simulink library "xbsIndex_r4"  (Simulink 7.1)
(part 4 of 9)

  Expression : S-Function  LoadFcn=xlBlockLoadCallback(gcbh);  FunctionName=sysgen  Parameters=ptable_  EnableBusSupport=off  mask(Xilinx Bitwise Expression Evaluator Block){expression=a & b, align_bp_sgadvanced=, align_bp=on, en_sgadvanced=, en=off, latency=0, precision_sgadvanced=, precision=Full, arith_type_sgadvanced=, arith_type=Unsigned, n_bits=16, bin_pt=0, dbl_ovrd_sgadvanced=, dbl_ovrd=off, xl_use_area_sgadvanced=, xl_use_area=off, xl_area=[0,0,0,0,0,0,0], has_advanced_control=0, sggui_pos=-1,-1,-1,-1, block_type=expr, block_version=, sg_icon_stat=65,60,2,1,white,blue,0,87655dbc,right,,[ ],[ ], sg_mask_display=|, sg_list_contents=, sg_blockgui_xml=}
      mask sg_mask_display=|
      | fprintf('','COMMENT: begin icon graphics');
      | patch([0 65 65 0 0 ],[0 0 60 60 0 ],[0.77 0.82 0.91 ]);
      | plot([0 65 65 0 0 ],[0 0 60 60 0 ]);
      | patch([14.2 25.76 33.76 41.76 49.76 33.76 22.2 14.2 ],[38.88 38.88 46.88 38.88 46.88 46.88 46.88 38.88 ],[1 1 1 ]);
      | patch([22.2 33.76 25.76 14.2 22.2 ],[30.88 30.88 38.88 38.88 30.88 ],[0.931 0.946 0.973 ]);
      | patch([14.2 25.76 33.76 22.2 14.2 ],[22.88 22.88 30.88 30.88 22.88 ],[1 1 1 ]);
      | patch([22.2 49.76 41.76 33.76 25.76 14.2 22.2 ],[14.88 14.88 22.88 14.88 22.88 22.88 14.88 ],[0.931 0.946 0.973 ]);
      | fprintf('','COMMENT: end icon graphics');
      | fprintf('','COMMENT: begin icon text');
      | color('black');port_label('input',1,'a');
      | color('black');port_label('input',2,'b');
      | color('black');port_label('output',1,'\bfa & b','texmode','on');
      | fprintf('','COMMENT: end icon text');
      mask prompts: align_bp_sgadvanced ""; align_bp "Align binary point"; en_sgadvanced ""; en "Provide enable port"; precision_sgadvanced ""; arith_type_sgadvanced ""; arith_type "Arithmetic type"; n_bits "Number of bits"; bin_pt "Binary point"; dbl_ovrd_sgadvanced ""; dbl_ovrd "Override with doubles"; xl_use_area_sgadvanced ""; xl_use_area "Define FPGA area for resource estimation"; xl_area "FPGA area [slices, FFs, BRAMs, LUTs, IOBs, emb. mults, TBUFs]"; has_advanced_control ""; sggui_pos ""; block_type ""; block_version ""; sg_icon_stat ""; sg_mask_display ""; sg_list_contents ""; sg_blockgui_xml ""
      mask help: Xilinx Bitwise Expression Evaluator
      mask init:
      | try
      |   tmp_gcb = gcb;
      |   tmp_gcbh = gcbh;
      |   if (strcmp('SysGenIndex',get_param(bdroot(tmp_gcbh),'tag')) && ~isempty(regexp(bdroot(tmp_gcb), '^xbs', 'once')))
      |     return;
      |   end;
      |   xlMungeMaskParams;
      |   block_config = 'sysgen_blockset:Expr_config';
      | 
      |   block_type='expr';
      | 
      |   serialized_declarations = '{''align_bp''=>''Int'',''arith_type''=>''Int'',''bin_pt''=>''Int'',''dbl_ovrd''=>''Int'',''en''=>''Int'',''expression''=>''String'',''inports''=>''String'',''latency''=>''Int'',''n_bits''=>''Int'',''period''=>''Double'',''precision''=>''Int'',''sim_engine''=>''Int'',''sysgen_root''=>''String'',''block_type''=>''String''}';
      |   xlexpr_init();
      |   ptable_ = xlblockprep(get_param(tmp_gcb, 'MaskWSVariables'));
      |   try
      |     xlBlockMoveCallback(tmp_gcbh);
      |   catch 
      |      clear global xl_updateicon_recursion_guard;
      |   end;
      | catch
      |   global dbgsysgen;
      |   if(~isempty(dbgsysgen) && dbgsysgen)
      |     e = regexprep(lasterr, '\n', '\nError: ');
      |     disp(['Error: While running MaskInit code on block ' tmp_gcb ': ' e]);
      |     error(e);
      |   end
      | end
      settings: CopyFcn=xlBlockMoveCallback(gcbh);  DeleteFcn=xlDestroyGui(gcbh);  ModelCloseFcn=xlDestroyGui(gcbh);  PreSaveFcn=xlBlockPreSaveCallback(gcbh);  PostSaveFcn=xlBlockPostSaveCallback(gcbh);  DestroyFcn=xlDestroyGui(gcbh);  OpenFcn=xlOpenGui(gcbh, 'expr_gui.xml', @xlmagicenablement, -1)  CloseFcn=xlDestroyGui(gcbh);  MoveFcn=xlBlockMoveCallback(gcbh);
      mask Help: eval('');xlDoc('-book','sysgen','-topic','Expression');
      mask StyleString: edit,edit,checkbox,edit,checkbox,edit,edit,popup(Full|User Defined),edit,popup(Signed  (2's comp)|Unsigned),edit,edit,edit,checkbox,edit,checkbox,edit,edit,edit,edit,edit,edit,edit,edit,edit
      mask Display:
      | fprintf('','COMMENT: begin icon graphics');
      | patch([0 65 65 0 0 ],[0 0 60 60 0 ],[0.77 0.82 0.91 ]);
      | plot([0 65 65 0 0 ],[0 0 60 60 0 ]);
      | patch([14.2 25.76 33.76 41.76 49.76 33.76 22.2 14.2 ],[38.88 38.88 46.88 38.88 46.88 46.88 46.88 38.88 ],[1 1 1 ]);
      | patch([22.2 33.76 25.76 14.2 22.2 ],[30.88 30.88 38.88 38.88 30.88 ],[0.931 0.946 0.973 ]);
      | patch([14.2 25.76 33.76 22.2 14.2 ],[22.88 22.88 30.88 30.88 22.88 ],[1 1 1 ]);
      | patch([22.2 49.76 41.76 33.76 25.76 14.2 22.2 ],[14.88 14.88 22.88 14.88 22.88 22.88 14.88 ],[0.931 0.946 0.973 ]);
      | fprintf('','COMMENT: end icon graphics');
      | fprintf('','COMMENT: begin icon text');
      | color('black');port_label('input',1,'a');
      | color('black');port_label('input',2,'b');
      | color('black');port_label('output',1,'\bfa & b','texmode','on');
      | fprintf('','COMMENT: end icon text');
  FDATool : S-Function  FunctionName=xlpermissive  Parameters=''  EnableBusSupport=off  mask(Xilinx FDATool Interface Block){infoedit=FDATool, ShowPortLabels=, has_advanced_control=0, sggui_pos=-1,-1,-1,-1, block_type=fdatool, block_version=, sg_icon_stat=54,56,-1,-1,blue,white,0,07734,right,,[ ],[ ], sg_mask_display=|, sg_list_contents=, sg_blockgui_xml=}
      mask sg_mask_display=|
      | fprintf('','COMMENT: begin icon graphics');
      | patch([0 54 54 0 0 ],[0 0 56 56 0 ],[1 1 1 ]);
      | plot([0 54 54 0 0 ],[0 0 56 56 0 ]);
      | patch([11.425 21.54 28.54 35.54 42.54 28.54 18.425 11.425 ],[35.77 35.77 42.77 35.77 42.77 42.77 42.77 35.77 ],[0.839 0.874 0.937 ]);
      | patch([18.425 28.54 21.54 11.425 18.425 ],[28.77 28.77 35.77 35.77 28.77 ],[0.77 0.82 0.91 ]);
      | patch([11.425 21.54 28.54 18.425 11.425 ],[21.77 21.77 28.77 28.77 21.77 ],[0.839 0.874 0.937 ]);
      | patch([18.425 42.54 35.54 28.54 21.54 11.425 18.425 ],[14.77 14.77 21.77 14.77 21.77 21.77 14.77 ],[0.77 0.82 0.91 ]);
      | fprintf('','COMMENT: end icon graphics');
      | fprintf('','COMMENT: begin icon text');
      | fprintf('','COMMENT: end icon text');plot(foox,foo);
      mask prompts: infoedit ""; ShowPortLabels ""; has_advanced_control ""; sggui_pos ""; block_type ""; block_version ""; sg_icon_stat ""; sg_mask_display ""; sg_list_contents ""; sg_blockgui_xml ""
      mask help: FDATool
      mask init:
      | try
      |   tmp_gcb = gcb;
      |   tmp_gcbh = gcbh;
      |   xlMungeMaskParams;
      | 
      |   block_type='fdatool';
      | 
      |   serialized_declarations = '{''block_type''=>''String''}';
      |   xlfdatool_init();
      |   ptable_ = xlblockprep(get_param(tmp_gcb, 'MaskWSVariables'));
      |   try
      |     xlBlockMoveCallback(tmp_gcbh);
      |   catch 
      |      clear global xl_updateicon_recursion_guard;
      |   end;
      | catch
      |   global dbgsysgen;
      |   if(~isempty(dbgsysgen) && dbgsysgen)
      |     e = regexprep(lasterr, '\n', '\nError: ');
      |     disp(['Error: While running MaskInit code on block ' tmp_gcb ': ' e]);
      |     error(e);
      |   end
      | end
      settings: CopyFcn=xlfdatool_utils('BlockCopy');  DeleteFcn=xlfdatool_utils('CloseFcn');  ModelCloseFcn=xlfdatool_utils('ModelCloseFcn');  NameChangeFcn=xlfdatool_utils('NameChange');  OpenFcn=xlfdatool_utils('OpenFcn');  CloseFcn=xlfdatool_utils('CloseFcn');  MoveFcn=xlBlockMoveCallback(gcbh);
      mask Help: eval('');xlDoc('-book','sysgen','-topic','FDATool');
      mask Display:
      | fprintf('','COMMENT: begin icon graphics');
      | patch([0 54 54 0 0 ],[0 0 56 56 0 ],[1 1 1 ]);
      | plot([0 54 54 0 0 ],[0 0 56 56 0 ]);
      | patch([11.425 21.54 28.54 35.54 42.54 28.54 18.425 11.425 ],[35.77 35.77 42.77 35.77 42.77 42.77 42.77 35.77 ],[0.839 0.874 0.937 ]);
      | patch([18.425 28.54 21.54 11.425 18.425 ],[28.77 28.77 35.77 35.77 28.77 ],[0.77 0.82 0.91 ]);
      | patch([11.425 21.54 28.54 18.425 11.425 ],[21.77 21.77 28.77 28.77 21.77 ],[0.839 0.874 0.937 ]);
      | patch([18.425 42.54 35.54 28.54 21.54 11.425 18.425 ],[14.77 14.77 21.77 14.77 21.77 21.77 14.77 ],[0.77 0.82 0.91 ]);
      | fprintf('','COMMENT: end icon graphics');
      | fprintf('','COMMENT: begin icon text');
      | fprintf('','COMMENT: end icon text');plot(foox,foo);
  "FFT v1_0 " : S-Function  LoadFcn=xlBlockLoadCallback(gcbh);  FunctionName=sysgen  Parameters=ptable_  EnableBusSupport=off  mask(Xilinx Fast Fourier Transform v1_0 Block){infoedit=Radix-4 Cooley-Tukey fast Fourier transform (FFT).  Supports 16, 64, 256, and 1024 point transforms on 16-bit data.<br><br>Devices Supported: Virtex, n_sgadvanced=, n=64, mem_sgadvanced=, mem=Triple, scale_mode_sgadvanced=, scale_mode=1/N, oflw_inv_sgadvanced=, oflw_inv=on, rst_sgadvanced=, rst=off, dbl_ovrd_sgadvanced=, dbl_ovrd=off, explicit_period_sgadvanced=, explicit_period=off, period=1, xl_use_area_sgadvanced=, xl_use_area=off, xl_area=[0,0,0,0,0,0,0], has_advanced_control=0, sggui_pos=-1,-1,-1,-1, block_type=fft, block_version=, sg_icon_stat=60,88,-1,-1,white,blue,0,07734,right,,[ ],[ ], sg_mask_display=|, sg_list_contents=, sg_blockgui_xml=}
      mask sg_mask_display=|
      | fprintf('','COMMENT: begin icon graphics');
      | patch([0 60 60 0 0 ],[0 0 88 88 0 ],[0.77 0.82 0.91 ]);
      | plot([0 60 60 0 0 ],[0 0 88 88 0 ]);
      | patch([12.2 23.76 31.76 39.76 47.76 31.76 20.2 12.2 ],[52.88 52.88 60.88 52.88 60.88 60.88 60.88 52.88 ],[1 1 1 ]);
      | patch([20.2 31.76 23.76 12.2 20.2 ],[44.88 44.88 52.88 52.88 44.88 ],[0.931 0.946 0.973 ]);
      | patch([12.2 23.76 31.76 20.2 12.2 ],[36.88 36.88 44.88 44.88 36.88 ],[1 1 1 ]);
      | patch([20.2 47.76 39.76 31.76 23.76 12.2 20.2 ],[28.88 28.88 36.88 28.88 36.88 36.88 28.88 ],[0.931 0.946 0.973 ]);
      | fprintf('','COMMENT: end icon graphics');
      | fprintf('','COMMENT: begin icon text');
      | fprintf('','COMMENT: end icon text');
      mask prompts: infoedit ""; n_sgadvanced ""; n "Number of sample points (N)"; mem_sgadvanced ""; mem "Memory usage"; scale_mode_sgadvanced ""; scale_mode "Scale output by"; oflw_inv_sgadvanced ""; oflw_inv "Invalidate transform on overflow"; rst_sgadvanced ""; rst "Provide synchronous reset port"; dbl_ovrd_sgadvanced ""; dbl_ovrd "Override with doubles"; explicit_period_sgadvanced ""; explicit_period "Specify explicit sample period"; period ""; xl_use_area_sgadvanced ""; xl_use_area "Define FPGA area for resource estimation"; xl_area "FPGA area [slices, FFs, BRAMs, LUTs, IOBs, emb. mults, TBUFs]"; has_advanced_control ""; sggui_pos ""; block_type ""; block_version ""; sg_icon_stat ""; sg_mask_display ""; sg_list_contents ""; sg_blockgui_xml ""
      mask help:
      | Radix-4 Cooley-Tukey fast Fourier transform (FFT).  Supports 16, 64, 256, and 1024 point transforms on 16-bit data.
      |
      | Devices Supported: Virtex
      mask init:
      | try
      |   tmp_gcb = gcb;
      |   tmp_gcbh = gcbh;
      |   if (strcmp('SysGenIndex',get_param(bdroot(tmp_gcbh),'tag')) && ~isempty(regexp(bdroot(tmp_gcb), '^xbs', 'once')))
      |     return;
      |   end;
      |   xlMungeMaskParams;
      |   block_config = 'sysgen_blockset:Removed_config';
      | 
      |   block_type='fft';
      | nport = get_param(gcbh, 'ports');
      | nin = nport(1);
      | nout = nport(2);
      | 
      |   serialized_declarations = '{''memory_usage''=>''Int'',''npts''=>''Int'',''oflw_inv''=>''Int'',''period''=>''Double'',''scale_mode''=>''Int'',''block_type''=>''String'',''nin''=>''Double'',''nout''=>''Double''}';
      |   xlfft_init();
      |   ptable_ = xlblockprep(get_param(tmp_gcb, 'MaskWSVariables'));
      |   try
      |     xlBlockMoveCallback(tmp_gcbh);
      |   catch 
      |      clear global xl_updateicon_recursion_guard;
      |   end;
      | catch
      |   global dbgsysgen;
      |   if(~isempty(dbgsysgen) && dbgsysgen)
      |     e = regexprep(lasterr, '\n', '\nError: ');
      |     disp(['Error: While running MaskInit code on block ' tmp_gcb ': ' e]);
      |     error(e);
      |   end
      | end
      settings: CopyFcn=xlBlockMoveCallback(gcbh);  DeleteFcn=xlDestroyGui(gcbh);  ModelCloseFcn=xlDestroyGui(gcbh);  PreSaveFcn=xlBlockPreSaveCallback(gcbh);  PostSaveFcn=xlBlockPostSaveCallback(gcbh);  DestroyFcn=xlDestroyGui(gcbh);  OpenFcn=xlOpenGui(gcbh, 'fft_gui.xml', @xlremovedenablement, -1)  CloseFcn=xlDestroyGui(gcbh);  MoveFcn=xlBlockMoveCallback(gcbh);
      mask Help: eval('');xlDoc('-book','sysgen','-topic','FFT_v1_0');
      mask StyleString: edit,edit,popup(16|64|256|1024),edit,popup(Single|Double|Triple),edit,popup(1/N|1/(2N)),edit,checkbox,edit,checkbox,edit,checkbox,edit,checkbox,edit,edit,checkbox,edit,edit,edit,edit,edit,edit,edit,edit,edit
      mask Display:
      | fprintf('','COMMENT: begin icon graphics');
      | patch([0 60 60 0 0 ],[0 0 88 88 0 ],[0.77 0.82 0.91 ]);
      | plot([0 60 60 0 0 ],[0 0 88 88 0 ]);
      | patch([12.2 23.76 31.76 39.76 47.76 31.76 20.2 12.2 ],[52.88 52.88 60.88 52.88 60.88 60.88 60.88 52.88 ],[1 1 1 ]);
      | patch([20.2 31.76 23.76 12.2 20.2 ],[44.88 44.88 52.88 52.88 44.88 ],[0.931 0.946 0.973 ]);
      | patch([12.2 23.76 31.76 20.2 12.2 ],[36.88 36.88 44.88 44.88 36.88 ],[1 1 1 ]);
      | patch([20.2 47.76 39.76 31.76 23.76 12.2 20.2 ],[28.88 28.88 36.88 28.88 36.88 36.88 28.88 ],[0.931 0.946 0.973 ]);
      | fprintf('','COMMENT: end icon graphics');
      | fprintf('','COMMENT: begin icon text');
      | fprintf('','COMMENT: end icon text');
  "FFT v3_1 " : S-Function  LoadFcn=xlBlockLoadCallback(gcbh);  FunctionName=sysgen  Parameters=ptable_  EnableBusSupport=off  mask(Xilinx Fast Fourier Transform v3_1 Block){infoedit=Devices Supported: Virtex-4, Virtex-II, Virtex-IIPro, Spartan-3 and Spartan-3E, arch_sgadvanced=, arch=Pipelined Streaming I/O, npts_sgadvanced=, npts=64, scaling_sgadvanced=, scaling=Unscaled, rounding_sgadvanced=, rounding=Truncation, tf_width_sgadvanced=, tf_width=8, en_n_sgadvanced=, en_n=off, has_ovflo_sgadvanced=, has_ovflo=off, rst_sgadvanced=, rst=off, en_sgadvanced=, en=off, op_order_sgadvanced=, op_order=Bit Reversed Order, dbl_ovrd_sgadvanced=, dbl_ovrd=off, explicit_period_sgadvanced=, explicit_period=off, period=1, use_dsp48_sgadvanced=, use_dsp48=off, twiddle_mem_type_sgadvanced=, twiddle_mem_type=Block RAM, data_mem_type_sgadvanced=, data_mem_type=Block RAM, num_bram_stages_sgadvanced=, num_bram_stages=3, xl_use_area_sgadvanced=, xl_use_area=off, xl_area=[0,0,0,0,0,0,0], has_advanced_control=0, sggui_pos=-1,-1,-1,-1, block_type=fftx, block_version=, sg_icon_stat=100,146,-1,-1,white,blue,0,07734,right,,[ ],[ ], sg_mask_display=|, sg_list_contents=, sg_blockgui_xml=}
      mask sg_mask_display=|
      | fprintf('','COMMENT: begin icon graphics');
      | patch([0 100 100 0 0 ],[0 0 146 146 0 ],[0.77 0.82 0.91 ]);
      | plot([0 100 100 0 0 ],[0 0 146 146 0 ]);
      | patch([18.85 39.08 53.08 67.08 81.08 53.08 32.85 18.85 ],[88.54 88.54 102.54 88.54 102.54 102.54 102.54 88.54 ],[1 1 1 ]);
      | patch([32.85 53.08 39.08 18.85 32.85 ],[74.54 74.54 88.54 88.54 74.54 ],[0.931 0.946 0.973 ]);
      | patch([18.85 39.08 53.08 32.85 18.85 ],[60.54 60.54 74.54 74.54 60.54 ],[1 1 1 ]);
      | patch([32.85 81.08 67.08 53.08 39.08 18.85 32.85 ],[46.54 46.54 60.54 46.54 60.54 60.54 46.54 ],[0.931 0.946 0.973 ]);
      | fprintf('','COMMENT: end icon graphics');
      | fprintf('','COMMENT: begin icon text');
      | fprintf('','COMMENT: end icon text');
      mask prompts: infoedit ""; arch_sgadvanced ""; arch "Implementation"; npts_sgadvanced ""; npts "Number of sample points"; scaling_sgadvanced ""; rounding_sgadvanced ""; rounding "Rounding mode"; tf_width_sgadvanced ""; tf_width "Phase factor bit width"; en_n_sgadvanced ""; en_n "Enable dynamic transform size"; has_ovflo_sgadvanced ""; has_ovflo "Provide overflow port"; rst_sgadvanced ""; rst "Provide synchronous reset port"; en_sgadvanced ""; en "Provide enable port"; op_order_sgadvanced ""; op_order "Output ordering"; dbl_ovrd_sgadvanced ""; dbl_ovrd "Override with doubles"; explicit_period_sgadvanced ""; explicit_period "Specify explicit sample period"; period ""; use_dsp48_sgadvanced ""; use_dsp48 "Optimize for speed using DSP48"; twiddle_mem_type_sgadvanced ""; twiddle_mem_type "Phase factor memory type"; data_mem_type_sgadvanced ""; data_mem_type "Data memory type"; num_bram_stages_sgadvanced ""; num_bram_stages "Number of stages using block RAM"; xl_use_area_sgadvanced ""; xl_use_area "Define FPGA area for resource estimation"; xl_area "FPGA area [slices, FFs, BRAMs, LUTs, IOBs, emb. mults, TBUFs]"; has_advanced_control ""; sggui_pos ""; block_type ""; block_version ""; sg_icon_stat ""; sg_mask_display ""; sg_list_contents ""; sg_blockgui_xml ""
      mask help: Devices Supported: Virtex-4, Virtex-II, Virtex-IIPro, Spartan-3 and Spartan-3E
      mask init:
      | try
      |   tmp_gcb = gcb;
      |   tmp_gcbh = gcbh;
      |   if (strcmp('SysGenIndex',get_param(bdroot(tmp_gcbh),'tag')) && ~isempty(regexp(bdroot(tmp_gcb), '^xbs', 'once')))
      |     return;
      |   end;
      |   xlMungeMaskParams;
      |   block_config = 'sysgen_blockset:Removed_config';
      | 
      |   block_type='fftx';
      | nport = get_param(gcbh, 'ports');
      | nin = nport(1);
      | nout = nport(2);
      | 
      |   serialized_declarations = '{''arch''=>''Int'',''c_family''=>''Int'',''data_mem_type''=>''Int'',''en''=>''Int'',''en_n''=>''Int'',''has_ovflo''=>''Int'',''npts''=>''Int'',''num_bram_stages''=>''Int'',''op_order''=>''Int'',''period''=>''Double'',''rounding''=>''Int'',''rst''=>''Int'',''scaling''=>''Int'',''tf_width''=>''Int'',''twiddle_mem_type''=>''Int'',''use_dsp48''=>''Int'',''xlISEVer''=>''String'',''xlv2fft_dll''=>''String'',''block_type''=>''String'',''nin''=>''Double'',''nout''=>''Double''}';
      |   xlfftx_init();
      |   ptable_ = xlblockprep(get_param(tmp_gcb, 'MaskWSVariables'));
      |   try
      |     xlBlockMoveCallback(tmp_gcbh);
      |   catch 
      |      clear global xl_updateicon_recursion_guard;
      |   end;
      | catch
      |   global dbgsysgen;
      |   if(~isempty(dbgsysgen) && dbgsysgen)
      |     e = regexprep(lasterr, '\n', '\nError: ');
      |     disp(['Error: While running MaskInit code on block ' tmp_gcb ': ' e]);
      |     error(e);
      |   end
      | end
      settings: CopyFcn=xlBlockMoveCallback(gcbh);  DeleteFcn=xlDestroyGui(gcbh);  ModelCloseFcn=xlDestroyGui(gcbh);  PreSaveFcn=xlBlockPreSaveCallback(gcbh);  PostSaveFcn=xlBlockPostSaveCallback(gcbh);  DestroyFcn=xlDestroyGui(gcbh);  OpenFcn=xlOpenGui(gcbh, 'fftx_gui.xml', @xlremovedenablement, -1)  CloseFcn=xlDestroyGui(gcbh);  MoveFcn=xlBlockMoveCallback(gcbh);
      mask Help: eval('');xlDoc('-book','sysgen','-topic','FFT_v3_1');
      mask StyleString: edit,edit,popup(Radix-4 Streaming I/O|Radix-4 Burst I/O|Radix-2 Minimum Resources|Pipelined Streaming I/O),edit,popup(8|16|32|64|128|256|512|1024|2048|4096|8192|16384|32768|65536),edit,popup(Unscaled|Scaled|Block Floating Point),edit,popup(Truncation|Convergent Rounding),edit,popup(8|12|16|20|24),edit,checkbox,edit,checkbox,edit,checkbox,edit,checkbox,edit,popup(Bit Reversed Order|Natural Order),edit,checkbox,edit,checkbox,edit,edit,checkbox,edit,popup(Block RAM|Distributed RAM),edit,popup(Block RAM|Distributed RAM),edit,popup(0|1|2|3|4|5|6|7|8|9|10|11|12|13),edit,checkbox,edit,edit,edit,edit,edit,edit,edit,edit,edit
      mask Display:
      | fprintf('','COMMENT: begin icon graphics');
      | patch([0 100 100 0 0 ],[0 0 146 146 0 ],[0.77 0.82 0.91 ]);
      | plot([0 100 100 0 0 ],[0 0 146 146 0 ]);
      | patch([18.85 39.08 53.08 67.08 81.08 53.08 32.85 18.85 ],[88.54 88.54 102.54 88.54 102.54 102.54 102.54 88.54 ],[1 1 1 ]);
      | patch([32.85 53.08 39.08 18.85 32.85 ],[74.54 74.54 88.54 88.54 74.54 ],[0.931 0.946 0.973 ]);
      | patch([18.85 39.08 53.08 32.85 18.85 ],[60.54 60.54 74.54 74.54 60.54 ],[1 1 1 ]);
      | patch([32.85 81.08 67.08 53.08 39.08 18.85 32.85 ],[46.54 46.54 60.54 46.54 60.54 60.54 46.54 ],[0.931 0.946 0.973 ]);
      | fprintf('','COMMENT: end icon graphics');
      | fprintf('','COMMENT: begin icon text');
      | fprintf('','COMMENT: end icon text');
  "FFT v3_2 " : S-Function  LoadFcn=xlBlockLoadCallback(gcbh);  FunctionName=sysgen  Parameters=ptable_  EnableBusSupport=off  mask(Xilinx Fast Fourier Transform v3_2 Block){infoedit=Devices Supported: Virtex-4, Virtex-II, Virtex-IIPro, Spartan-3 and Spartan-3E, arch_sgadvanced=, arch=Pipelined Streaming I/O, npts_sgadvanced=, npts=1024, op_order_sgadvanced=, op_order=Natural Order, scaling_sgadvanced=, scaling=Unscaled, rounding_sgadvanced=, rounding=Truncation, tf_width_sgadvanced=, tf_width=8, en_n_sgadvanced=, en_n=off, has_ovflo_sgadvanced=, has_ovflo=off, rst_sgadvanced=, rst=off, en_sgadvanced=, en=off, dbl_ovrd_sgadvanced=, dbl_ovrd=off, use_dsp48_bfly_sgadvanced=, use_dsp48_bfly=off, use_dsp48_cmpy_sgadvanced=, use_dsp48_cmpy=off, use_dsp48_sincos_sgadvanced=, use_dsp48_sincos=off, twiddle_mem_type_sgadvanced=, twiddle_mem_type=Block RAM, data_mem_type_sgadvanced=, data_mem_type=Block RAM, num_bram_stages_sgadvanced=, num_bram_stages=3, xl_use_area_sgadvanced=, xl_use_area=off, xl_area=[0,0,0,0,0,0,0], explicit_period=, period=1, has_advanced_control=0, sggui_pos=-1,-1,-1,-1, block_type=fftv32, block_version=, sg_icon_stat=100,146,-1,-1,white,blue,0,07734,right,,[ ],[ ], sg_mask_display=|, sg_list_contents=, sg_blockgui_xml=}
      mask sg_mask_display=|
      | fprintf('','COMMENT: begin icon graphics');
      | patch([0 100 100 0 0 ],[0 0 146 146 0 ],[0.77 0.82 0.91 ]);
      | plot([0 100 100 0 0 ],[0 0 146 146 0 ]);
      | patch([18.85 39.08 53.08 67.08 81.08 53.08 32.85 18.85 ],[88.54 88.54 102.54 88.54 102.54 102.54 102.54 88.54 ],[1 1 1 ]);
      | patch([32.85 53.08 39.08 18.85 32.85 ],[74.54 74.54 88.54 88.54 74.54 ],[0.931 0.946 0.973 ]);
      | patch([18.85 39.08 53.08 32.85 18.85 ],[60.54 60.54 74.54 74.54 60.54 ],[1 1 1 ]);
      | patch([32.85 81.08 67.08 53.08 39.08 18.85 32.85 ],[46.54 46.54 60.54 46.54 60.54 60.54 46.54 ],[0.931 0.946 0.973 ]);
      | fprintf('','COMMENT: end icon graphics');
      | fprintf('','COMMENT: begin icon text');
      | fprintf('','COMMENT: end icon text');
      mask prompts: infoedit ""; arch_sgadvanced ""; arch "Implementation"; npts_sgadvanced ""; npts "Number of sample points"; op_order_sgadvanced ""; op_order "Output ordering"; scaling_sgadvanced ""; rounding_sgadvanced ""; rounding "Rounding mode"; tf_width_sgadvanced ""; tf_width "Phase factor bit width"; en_n_sgadvanced ""; en_n "Enable dynamic transform size"; has_ovflo_sgadvanced ""; has_ovflo "Provide overflow port"; rst_sgadvanced ""; rst "Provide synchronous reset port"; en_sgadvanced ""; en "Provide enable port"; dbl_ovrd_sgadvanced ""; dbl_ovrd "Override with doubles"; use_dsp48_bfly_sgadvanced ""; use_dsp48_bfly "Butterfly arithmetic"; use_dsp48_cmpy_sgadvanced ""; use_dsp48_cmpy "Complex multiplication"; use_dsp48_sincos_sgadvanced ""; use_dsp48_sincos "Phase factor generation"; twiddle_mem_type_sgadvanced ""; twiddle_mem_type "Phase factor memory type"; data_mem_type_sgadvanced ""; data_mem_type "Data memory type"; num_bram_stages_sgadvanced ""; num_bram_stages "Number of stages using block RAM"; xl_use_area_sgadvanced ""; xl_use_area "Define FPGA area for resource estimation"; xl_area "FPGA area [slices, FFs, BRAMs, LUTs, IOBs, emb. mults, TBUFs]"; explicit_period ""; period ""; has_advanced_control ""; sggui_pos ""; block_type ""; block_version ""; sg_icon_stat ""; sg_mask_display ""; sg_list_contents ""; sg_blockgui_xml ""
      mask help: Devices Supported: Virtex-4, Virtex-II, Virtex-IIPro, Spartan-3 and Spartan-3E
      mask init:
      | try
      |   tmp_gcb = gcb;
      |   tmp_gcbh = gcbh;
      |   if (strcmp('SysGenIndex',get_param(bdroot(tmp_gcbh),'tag')) && ~isempty(regexp(bdroot(tmp_gcb), '^xbs', 'once')))
      |     return;
      |   end;
      |   xlMungeMaskParams;
      |   block_config = 'sysgen_blockset:Removed_config';
      | 
      |   block_type='fftv32';
      | nport = get_param(gcbh, 'ports');
      | nin = nport(1);
      | nout = nport(2);
      | 
      |   serialized_declarations = '{''arch''=>''Int'',''c_family''=>''Int'',''data_mem_type''=>''Int'',''en''=>''Int'',''en_n''=>''Int'',''has_ovflo''=>''Int'',''npts''=>''Int'',''num_bram_stages''=>''Int'',''op_order''=>''Int'',''rounding''=>''Int'',''rst''=>''Int'',''scaling''=>''Int'',''tf_width''=>''Int'',''twiddle_mem_type''=>''Int'',''use_dsp48_bfly''=>''Int'',''use_dsp48_cmpy''=>''Int'',''use_dsp48_sincos''=>''Int'',''xlISEVer''=>''String'',''xlv3fft_dll''=>''String'',''block_type''=>''String'',''nin''=>''Double'',''nout''=>''Double''}';
      |   xlfftv32_init();
      |   ptable_ = xlblockprep(get_param(tmp_gcb, 'MaskWSVariables'));
      |   try
      |     xlBlockMoveCallback(tmp_gcbh);
      |   catch 
      |      clear global xl_updateicon_recursion_guard;
      |   end;
      | catch
      |   global dbgsysgen;
      |   if(~isempty(dbgsysgen) && dbgsysgen)
      |     e = regexprep(lasterr, '\n', '\nError: ');
      |     disp(['Error: While running MaskInit code on block ' tmp_gcb ': ' e]);
      |     error(e);
      |   end
      | end
      settings: CopyFcn=xlBlockMoveCallback(gcbh);  DeleteFcn=xlDestroyGui(gcbh);  ModelCloseFcn=xlDestroyGui(gcbh);  PreSaveFcn=xlBlockPreSaveCallback(gcbh);  PostSaveFcn=xlBlockPostSaveCallback(gcbh);  DestroyFcn=xlDestroyGui(gcbh);  OpenFcn=xlOpenGui(gcbh, 'fftv32_gui.xml', @xlremovedenablement, -1)  CloseFcn=xlDestroyGui(gcbh);  MoveFcn=xlBlockMoveCallback(gcbh);
      mask Help: eval('');xlDoc('-book','sysgen','-topic','FFT_v3_2');
      mask StyleString: edit,edit,popup(Radix-4 Burst I/O|Radix-2 Minimum Resources|Pipelined Streaming I/O),edit,popup(8|16|32|64|128|256|512|1024|2048|4096|8192|16384|32768|65536),edit,popup(Bit Reversed Order|Natural Order),edit,popup(Unscaled|Scaled|Block Floating Point),edit,popup(Truncation|Convergent Rounding),edit,popup(8|9|10|11|12|13|14|15|16|17|18|19|20|21|22|23|24),edit,checkbox,edit,checkbox,edit,checkbox,edit,checkbox,edit,checkbox,edit,checkbox,edit,checkbox,edit,checkbox,edit,popup(Block RAM|Distributed RAM),edit,popup(Block RAM|Distributed RAM),edit,popup(0|1|2|3|4|5|6|7|8|9|10|11|12|13),edit,checkbox,edit,edit,edit,edit,edit,edit,edit,edit,edit,edit,edit
      mask Display:
      | fprintf('','COMMENT: begin icon graphics');
      | patch([0 100 100 0 0 ],[0 0 146 146 0 ],[0.77 0.82 0.91 ]);
      | plot([0 100 100 0 0 ],[0 0 146 146 0 ]);
      | patch([18.85 39.08 53.08 67.08 81.08 53.08 32.85 18.85 ],[88.54 88.54 102.54 88.54 102.54 102.54 102.54 88.54 ],[1 1 1 ]);
      | patch([32.85 53.08 39.08 18.85 32.85 ],[74.54 74.54 88.54 88.54 74.54 ],[0.931 0.946 0.973 ]);
      | patch([18.85 39.08 53.08 32.85 18.85 ],[60.54 60.54 74.54 74.54 60.54 ],[1 1 1 ]);
      | patch([32.85 81.08 67.08 53.08 39.08 18.85 32.85 ],[46.54 46.54 60.54 46.54 60.54 60.54 46.54 ],[0.931 0.946 0.973 ]);
      | fprintf('','COMMENT: end icon graphics');
      | fprintf('','COMMENT: begin icon text');
      | fprintf('','COMMENT: end icon text');
  "FFT v4_1 " : S-Function  LoadFcn=xlBlockLoadCallback(gcbh);  FunctionName=sysgen  Parameters=ptable_  EnableBusSupport=off  mask(Xilinx Fast Fourier Transform v4_1 Block){infoedit=Devices Supported: Virtex-5, Virtex-4, Virtex-IIPro, Spartan-3, Spartan-3A and Spartan-3E, arch_sgadvanced=, arch=Pipelined Streaming I/O, npts_sgadvanced=, npts=1024, op_order_sgadvanced=, op_order=Natural Order, scaling_sgadvanced=, scaling=Unscaled, rounding_sgadvanced=, rounding=Truncation, tf_width_sgadvanced=, tf_width=8, en_n_sgadvanced=, en_n=off, has_ovflo_sgadvanced=, has_ovflo=off, rst_sgadvanced=, rst=off, en_sgadvanced=, en=off, dbl_ovrd_sgadvanced=, dbl_ovrd=off, use_dsp48_bfly_sgadvanced=, use_dsp48_bfly=off, use_dsp48_cmpy_sgadvanced=, use_dsp48_cmpy=off, twiddle_mem_type_sgadvanced=, twiddle_mem_type=Block RAM, data_mem_type_sgadvanced=, data_mem_type=Block RAM, num_bram_stages_sgadvanced=, num_bram_stages=3, xl_use_area_sgadvanced=, xl_use_area=off, xl_area=[0,0,0,0,0,0,0], explicit_period=, period=1, has_advanced_control=0, sggui_pos=-1,-1,-1,-1, block_type=fftv41, block_version=, sg_icon_stat=100,146,-1,-1,white,blue,0,07734,right,,[ ],[ ], sg_mask_display=|, sg_list_contents=, sg_blockgui_xml=}
      mask sg_mask_display=|
      | fprintf('','COMMENT: begin icon graphics');
      | patch([0 100 100 0 0 ],[0 0 146 146 0 ],[0.77 0.82 0.91 ]);
      | plot([0 100 100 0 0 ],[0 0 146 146 0 ]);
      | patch([18.85 39.08 53.08 67.08 81.08 53.08 32.85 18.85 ],[88.54 88.54 102.54 88.54 102.54 102.54 102.54 88.54 ],[1 1 1 ]);
      | patch([32.85 53.08 39.08 18.85 32.85 ],[74.54 74.54 88.54 88.54 74.54 ],[0.931 0.946 0.973 ]);
      | patch([18.85 39.08 53.08 32.85 18.85 ],[60.54 60.54 74.54 74.54 60.54 ],[1 1 1 ]);
      | patch([32.85 81.08 67.08 53.08 39.08 18.85 32.85 ],[46.54 46.54 60.54 46.54 60.54 60.54 46.54 ],[0.931 0.946 0.973 ]);
      | fprintf('','COMMENT: end icon graphics');
      | fprintf('','COMMENT: begin icon text');
      | fprintf('','COMMENT: end icon text');
      mask prompts: infoedit ""; arch_sgadvanced ""; arch "Implementation"; npts_sgadvanced ""; npts "Number of sample points"; op_order_sgadvanced ""; op_order "Output ordering"; scaling_sgadvanced ""; rounding_sgadvanced ""; rounding "Rounding mode"; tf_width_sgadvanced ""; tf_width "Phase factor bit width"; en_n_sgadvanced ""; en_n "Enable dynamic transform size"; has_ovflo_sgadvanced ""; has_ovflo "Provide overflow port"; rst_sgadvanced ""; rst "Provide synchronous reset port"; en_sgadvanced ""; en "Provide enable port"; dbl_ovrd_sgadvanced ""; dbl_ovrd "Override with doubles"; use_dsp48_bfly_sgadvanced ""; use_dsp48_bfly "Butterfly arithmetic"; use_dsp48_cmpy_sgadvanced ""; use_dsp48_cmpy "Complex multiplication"; twiddle_mem_type_sgadvanced ""; twiddle_mem_type "Phase factor memory type"; data_mem_type_sgadvanced ""; data_mem_type "Data memory type"; num_bram_stages_sgadvanced ""; num_bram_stages "Number of stages using block RAM"; xl_use_area_sgadvanced ""; xl_use_area "Define FPGA area for resource estimation"; xl_area "FPGA area [slices, FFs, BRAMs, LUTs, IOBs, emb. mults, TBUFs]"; explicit_period ""; period ""; has_advanced_control ""; sggui_pos ""; block_type ""; block_version ""; sg_icon_stat ""; sg_mask_display ""; sg_list_contents ""; sg_blockgui_xml ""
      mask help: Devices Supported: Virtex-5, Virtex-4, Virtex-IIPro, Spartan-3, Spartan-3A and Spartan-3E
      mask init:
      | try
      |   tmp_gcb = gcb;
      |   tmp_gcbh = gcbh;
      |   if (strcmp('SysGenIndex',get_param(bdroot(tmp_gcbh),'tag')) && ~isempty(regexp(bdroot(tmp_gcb), '^xbs', 'once')))
      |     return;
      |   end;
      |   xlMungeMaskParams;
      |   block_config = 'sysgen_blockset:Removed_config';
      | 
      |   block_type='fftv41';
      | nport = get_param(gcbh, 'ports');
      | nin = nport(1);
      | nout = nport(2);
      | 
      |   serialized_declarations = '{''arch''=>''Int'',''c_family''=>''Int'',''data_mem_type''=>''Int'',''en''=>''Int'',''en_n''=>''Int'',''has_ovflo''=>''Int'',''npts''=>''Int'',''num_bram_stages''=>''Int'',''op_order''=>''Int'',''rounding''=>''Int'',''rst''=>''Int'',''scaling''=>''Int'',''tf_width''=>''Int'',''twiddle_mem_type''=>''Int'',''use_dsp48_bfly''=>''Int'',''use_dsp48_cmpy''=>''Int'',''xlISEVer''=>''String'',''xlv4fft_dll''=>''String'',''block_type''=>''String'',''nin''=>''Double'',''nout''=>''Double''}';
      |   xlfftv41_init();
      |   ptable_ = xlblockprep(get_param(tmp_gcb, 'MaskWSVariables'));
      |   try
      |     xlBlockMoveCallback(tmp_gcbh);
      |   catch 
      |      clear global xl_updateicon_recursion_guard;
      |   end;
      | catch
      |   global dbgsysgen;
      |   if(~isempty(dbgsysgen) && dbgsysgen)
      |     e = regexprep(lasterr, '\n', '\nError: ');
      |     disp(['Error: While running MaskInit code on block ' tmp_gcb ': ' e]);
      |     error(e);
      |   end
      | end
      settings: CopyFcn=xlBlockMoveCallback(gcbh);  DeleteFcn=xlDestroyGui(gcbh);  ModelCloseFcn=xlDestroyGui(gcbh);  PreSaveFcn=xlBlockPreSaveCallback(gcbh);  PostSaveFcn=xlBlockPostSaveCallback(gcbh);  DestroyFcn=xlDestroyGui(gcbh);  OpenFcn=xlOpenGui(gcbh, 'fftv41_gui.xml', @xlremovedenablement, -1)  CloseFcn=xlDestroyGui(gcbh);  MoveFcn=xlBlockMoveCallback(gcbh);
      mask Help: eval('');xlDoc('-book','sysgen','-topic','FFT_v4_1');
      mask StyleString: edit,edit,popup(Radix-4 Burst I/O|Radix-2 Burst I/O|Pipelined Streaming I/O|Radix-2 Lite Burst I/O),edit,popup(8|16|32|64|128|256|512|1024|2048|4096|8192|16384|32768|65536),edit,popup(Bit Reversed Order|Natural Order),edit,popup(Unscaled|Scaled|Block Floating Point),edit,popup(Truncation|Convergent Rounding),edit,popup(8|9|10|11|12|13|14|15|16|17|18|19|20|21|22|23|24),edit,checkbox,edit,checkbox,edit,checkbox,edit,checkbox,edit,checkbox,edit,checkbox,edit,checkbox,edit,popup(Block RAM|Distributed RAM),edit,popup(Block RAM|Distributed RAM),edit,popup(0|1|2|3|4|5|6|7|8|9|10|11|12|13),edit,checkbox,edit,edit,edit,edit,edit,edit,edit,edit,edit,edit,edit
      mask Display:
      | fprintf('','COMMENT: begin icon graphics');
      | patch([0 100 100 0 0 ],[0 0 146 146 0 ],[0.77 0.82 0.91 ]);
      | plot([0 100 100 0 0 ],[0 0 146 146 0 ]);
      | patch([18.85 39.08 53.08 67.08 81.08 53.08 32.85 18.85 ],[88.54 88.54 102.54 88.54 102.54 102.54 102.54 88.54 ],[1 1 1 ]);
      | patch([32.85 53.08 39.08 18.85 32.85 ],[74.54 74.54 88.54 88.54 74.54 ],[0.931 0.946 0.973 ]);
      | patch([18.85 39.08 53.08 32.85 18.85 ],[60.54 60.54 74.54 74.54 60.54 ],[1 1 1 ]);
      | patch([32.85 81.08 67.08 53.08 39.08 18.85 32.85 ],[46.54 46.54 60.54 46.54 60.54 60.54 46.54 ],[0.931 0.946 0.973 ]);
      | fprintf('','COMMENT: end icon graphics');
      | fprintf('','COMMENT: begin icon text');
      | fprintf('','COMMENT: end icon text');
  "FFT v5_0 " : S-Function  LoadFcn=xlBlockLoadCallback(gcbh);  FunctionName=sysgen  Parameters=ptable_  EnableBusSupport=off  mask(Xilinx Fast Fourier Transform v5_0 Block){infoedit=Devices Supported: Virtex-5, Virtex-4, Virtex-IIPro, Spartan-3, Spartan-3A and Spartan-3E, arch_sgadvanced=, arch=Pipelined Streaming I/O, npts_sgadvanced=, npts=1024, op_order_sgadvanced=, op_order=Natural Order, scaling_sgadvanced=, scaling=Unscaled, rounding_sgadvanced=, rounding=Truncation, tf_width_sgadvanced=, tf_width=8, cyclic_prefix_insertion_sgadvanced=, cyclic_prefix_insertion=off, en_n_sgadvanced=, en_n=off, has_ovflo_sgadvanced=, has_ovflo=off, rst_sgadvanced=, rst=off, en_sgadvanced=, en=off, dbl_ovrd_sgadvanced=, dbl_ovrd=off, use_dsp48_bfly_sgadvanced=, use_dsp48_bfly=off, use_dsp48_cmpy_sgadvanced=, use_dsp48_cmpy=off, twiddle_mem_type_sgadvanced=, twiddle_mem_type=Block RAM, data_mem_type_sgadvanced=, data_mem_type=Block RAM, num_bram_stages_sgadvanced=, num_bram_stages=3, xl_use_area_sgadvanced=, xl_use_area=off, xl_area=[0,0,0,0,0,0,0], has_advanced_control=0, sggui_pos=-1,-1,-1,-1, block_type=fftv5, block_version=, sg_icon_stat=100,146,-1,-1,white,blue,0,07734,right,,[ ],[ ], sg_mask_display=|, sg_list_contents=, sg_blockgui_xml=}
      mask sg_mask_display=|
      | fprintf('','COMMENT: begin icon graphics');
      | patch([0 100 100 0 0 ],[0 0 146 146 0 ],[0.77 0.82 0.91 ]);
      | plot([0 100 100 0 0 ],[0 0 146 146 0 ]);
      | patch([18.85 39.08 53.08 67.08 81.08 53.08 32.85 18.85 ],[88.54 88.54 102.54 88.54 102.54 102.54 102.54 88.54 ],[1 1 1 ]);
      | patch([32.85 53.08 39.08 18.85 32.85 ],[74.54 74.54 88.54 88.54 74.54 ],[0.931 0.946 0.973 ]);
      | patch([18.85 39.08 53.08 32.85 18.85 ],[60.54 60.54 74.54 74.54 60.54 ],[1 1 1 ]);
      | patch([32.85 81.08 67.08 53.08 39.08 18.85 32.85 ],[46.54 46.54 60.54 46.54 60.54 60.54 46.54 ],[0.931 0.946 0.973 ]);
      | fprintf('','COMMENT: end icon graphics');
      | fprintf('','COMMENT: begin icon text');
      | fprintf('','COMMENT: end icon text');
      mask prompts: infoedit ""; arch_sgadvanced ""; arch "Implementation"; npts_sgadvanced ""; npts "Number of sample points"; op_order_sgadvanced ""; op_order "Output ordering"; scaling_sgadvanced ""; rounding_sgadvanced ""; rounding "Rounding mode"; tf_width_sgadvanced ""; tf_width "Phase factor bit width"; cyclic_prefix_insertion_sgadvanced ""; cyclic_prefix_insertion "Cyclic prefix insertion"; en_n_sgadvanced ""; en_n "Enable dynamic transform size"; has_ovflo_sgadvanced ""; has_ovflo "Provide overflow port"; rst_sgadvanced ""; rst "Provide synchronous reset port"; en_sgadvanced ""; en "Provide enable port"; dbl_ovrd_sgadvanced ""; dbl_ovrd "Override with doubles"; use_dsp48_bfly_sgadvanced ""; use_dsp48_bfly "Butterfly arithmetic"; use_dsp48_cmpy_sgadvanced ""; use_dsp48_cmpy "Complex multiplication"; twiddle_mem_type_sgadvanced ""; twiddle_mem_type "Phase factor memory type"; data_mem_type_sgadvanced ""; data_mem_type "Data memory type"; num_bram_stages_sgadvanced ""; num_bram_stages "Number of stages using block RAM"; xl_use_area_sgadvanced ""; xl_use_area "Define FPGA area for resource estimation"; xl_area "FPGA area [slices, FFs, BRAMs, LUTs, IOBs, emb. mults, TBUFs]"; has_advanced_control ""; sggui_pos ""; block_type ""; block_version ""; sg_icon_stat ""; sg_mask_display ""; sg_list_contents ""; sg_blockgui_xml ""
      mask help: Devices Supported: Virtex-5, Virtex-4, Virtex-IIPro, Spartan-3, Spartan-3A and Spartan-3E
      mask init:
      | try
      |   tmp_gcb = gcb;
      |   tmp_gcbh = gcbh;
      |   if (strcmp('SysGenIndex',get_param(bdroot(tmp_gcbh),'tag')) && ~isempty(regexp(bdroot(tmp_gcb), '^xbs', 'once')))
      |     return;
      |   end;
      |   xlMungeMaskParams;
      |   block_config = 'sysgen_blockset:Removed_config';
      | 
      |   block_type='fftv5';
      | nport = get_param(gcbh, 'ports');
      | nin = nport(1);
      | nout = nport(2);
      | 
      |   serialized_declarations = '{''arch''=>''Int'',''cyclic_prefix_insertion''=>''Int'',''data_mem_type''=>''Int'',''en''=>''Int'',''en_n''=>''Int'',''has_ovflo''=>''Int'',''npts''=>''Int'',''num_bram_stages''=>''Int'',''op_order''=>''Int'',''rounding''=>''Int'',''rst''=>''Int'',''scaling''=>''Int'',''tf_width''=>''Int'',''twiddle_mem_type''=>''Int'',''use_dsp48_bfly''=>''Int'',''use_dsp48_cmpy''=>''Int'',''block_type''=>''String'',''nin''=>''Double'',''nout''=>''Double''}';
      |   ptable_ = xlblockprep(get_param(tmp_gcb, 'MaskWSVariables'));
      |   try
      |     xlBlockMoveCallback(tmp_gcbh);
      |   catch 
      |      clear global xl_updateicon_recursion_guard;
      |   end;
      | catch
      |   global dbgsysgen;
      |   if(~isempty(dbgsysgen) && dbgsysgen)
      |     e = regexprep(lasterr, '\n', '\nError: ');
      |     disp(['Error: While running MaskInit code on block ' tmp_gcb ': ' e]);
      |     error(e);
      |   end
      | end
      settings: CopyFcn=xlBlockMoveCallback(gcbh);  DeleteFcn=xlDestroyGui(gcbh);  ModelCloseFcn=xlDestroyGui(gcbh);  PreSaveFcn=xlBlockPreSaveCallback(gcbh);  PostSaveFcn=xlBlockPostSaveCallback(gcbh);  DestroyFcn=xlDestroyGui(gcbh);  OpenFcn=xlOpenGui(gcbh, 'fftv5_gui.xml', @xlremovedenablement, -1)  CloseFcn=xlDestroyGui(gcbh);  MoveFcn=xlBlockMoveCallback(gcbh);
      mask Help: eval('');xlDoc('-book','sysgen','-topic','FFT_v5_0');
      mask StyleString: edit,edit,popup(Radix-4 Burst I/O|Radix-2 Burst I/O|Pipelined Streaming I/O|Radix-2 Lite Burst I/O),edit,popup(8|16|32|64|128|256|512|1024|2048|4096|8192|16384|32768|65536),edit,popup(Bit Reversed Order|Natural Order),edit,popup(Unscaled|Scaled|Block Floating Point),edit,popup(Truncation|Convergent Rounding),edit,popup(8|9|10|11|12|13|14|15|16|17|18|19|20|21|22|23|24),edit,checkbox,edit,checkbox,edit,checkbox,edit,checkbox,edit,checkbox,edit,checkbox,edit,checkbox,edit,checkbox,edit,popup(Block RAM|Distributed RAM),edit,popup(Block RAM|Distributed RAM),edit,popup(0|1|2|3|4|5|6|7|8|9|10|11|12|13),edit,checkbox,edit,edit,edit,edit,edit,edit,edit,edit,edit
      mask Display:
      | fprintf('','COMMENT: begin icon graphics');
      | patch([0 100 100 0 0 ],[0 0 146 146 0 ],[0.77 0.82 0.91 ]);
      | plot([0 100 100 0 0 ],[0 0 146 146 0 ]);
      | patch([18.85 39.08 53.08 67.08 81.08 53.08 32.85 18.85 ],[88.54 88.54 102.54 88.54 102.54 102.54 102.54 88.54 ],[1 1 1 ]);
      | patch([32.85 53.08 39.08 18.85 32.85 ],[74.54 74.54 88.54 88.54 74.54 ],[0.931 0.946 0.973 ]);
      | patch([18.85 39.08 53.08 32.85 18.85 ],[60.54 60.54 74.54 74.54 60.54 ],[1 1 1 ]);
      | patch([32.85 81.08 67.08 53.08 39.08 18.85 32.85 ],[46.54 46.54 60.54 46.54 60.54 60.54 46.54 ],[0.931 0.946 0.973 ]);
      | fprintf('','COMMENT: end icon graphics');
      | fprintf('','COMMENT: begin icon text');
      | fprintf('','COMMENT: end icon text');
  FIFO : S-Function  LoadFcn=xlBlockLoadCallback(gcbh);  FunctionName=sysgen  Parameters=ptable_  EnableBusSupport=off  mask(Xilinx FIFO Block Block){performance_options_sgadvanced=, performance_options=Standard_FIFO, depth_sgadvanced=, depth=16, percent_nbits_sgadvanced=, percent_nbits=1, rst_sgadvanced=, rst=off, en_sgadvanced=, en=off, use_dcount_sgadvanced=, use_dcount=off, use_percent_full_port_sgadvanced=, use_percent_full_port=on, use_almost_empty_sgadvanced=, use_almost_empty=off, almost_empty_thresh=2, use_almost_full_sgadvanced=, use_almost_full=off, almost_full_thresh=14, dbl_ovrd_sgadvanced=, dbl_ovrd=off, mem_type_sgadvanced=, mem_type=Block RAM, xl_use_area_sgadvanced=, xl_use_area=off, xl_area=[0,0,0,0,0,0,0], infoedit=, almost_empty_offset=, almost_full_offset=, explicit_period=off, period=, store_only_valid=, init_zero=, xlcconfig=, has_advanced_control=0, sggui_pos=-1,-1,-1,-1, block_type=fifo, block_version=, sg_icon_stat=80,114,3,4,white,blue,0,2152acb9,right,,[ ],[ ], sg_mask_display=|, sg_list_contents=, sg_blockgui_xml=}
      mask sg_mask_display=|
      | fprintf('','COMMENT: begin icon graphics');
      | patch([0 80 80 0 0 ],[0 0 114 114 0 ],[0.77 0.82 0.91 ]);
      | plot([0 80 80 0 0 ],[0 0 114 114 0 ]);
      | patch([15.525 31.42 42.42 53.42 64.42 42.42 26.525 15.525 ],[69.21 69.21 80.21 69.21 80.21 80.21 80.21 69.21 ],[1 1 1 ]);
      | patch([26.525 42.42 31.42 15.525 26.525 ],[58.21 58.21 69.21 69.21 58.21 ],[0.931 0.946 0.973 ]);
      | patch([15.525 31.42 42.42 26.525 15.525 ],[47.21 47.21 58.21 58.21 47.21 ],[1 1 1 ]);
      | patch([26.525 64.42 53.42 42.42 31.42 15.525 26.525 ],[36.21 36.21 47.21 36.21 47.21 47.21 36.21 ],[0.931 0.946 0.973 ]);
      | fprintf('','COMMENT: end icon graphics');
      | fprintf('','COMMENT: begin icon text');
      | color('black');port_label('input',1,'din');
      | color('black');port_label('input',2,'we');
      | color('black');port_label('input',3,'re');
      | color('black');port_label('output',1,'dout');
      | color('black');port_label('output',2,'empty');
      | color('black');port_label('output',3,'%full');
      | color('black');port_label('output',4,'full');
      | fprintf('','COMMENT: end icon text');
      mask prompts: performance_options_sgadvanced ""; performance_options "Performance Options"; depth_sgadvanced ""; percent_nbits_sgadvanced ""; percent_nbits "Bits of precision to use for <tt>%full</tt> signal"; rst_sgadvanced ""; rst "Provide reset port"; en_sgadvanced ""; en "Provide enable port"; use_dcount_sgadvanced ""; use_dcount "Provide data count port"; use_percent_full_port_sgadvanced ""; use_percent_full_port "Provide percent full port"; use_almost_empty_sgadvanced ""; use_almost_empty "Provide almost empty port"; almost_empty_thresh "Almost empty threshold"; use_almost_full_sgadvanced ""; use_almost_full "Provide almost full port"; almost_full_thresh "Almost full threshold"; dbl_ovrd_sgadvanced ""; dbl_ovrd "Override with doubles"; mem_type_sgadvanced ""; mem_type "Memory Type"; xl_use_area_sgadvanced ""; xl_use_area "Define FPGA area for resource estimation"; xl_area "FPGA area [slices, FFs, BRAMs, LUTs, IOBs, emb. mults, TBUFs]"; infoedit ""; almost_empty_offset ""; almost_full_offset ""; explicit_period ""; period ""; store_only_valid ""; init_zero ""; xlcconfig ""; has_advanced_control ""; sggui_pos ""; block_type ""; block_version ""; sg_icon_stat ""; sg_mask_display ""; sg_list_contents ""; sg_blockgui_xml ""
      mask help: Xilinx FIFO Block
      mask init:
      | try
      |   tmp_gcb = gcb;
      |   tmp_gcbh = gcbh;
      |   if (strcmp('SysGenIndex',get_param(bdroot(tmp_gcbh),'tag')) && ~isempty(regexp(bdroot(tmp_gcb), '^xbs', 'once')))
      |     return;
      |   end;
      |   xlMungeMaskParams;
      |   block_config = 'sysgen_blockset:FIFO_config';
      | 
      |   block_type='fifo';
      | 
      |   serialized_declarations = '{''almost_empty_thresh''=>''Int'',''almost_full_thresh''=>''Int'',''depth''=>''Int'',''en''=>''Bool'',''explicit_period''=>''String'',''mem_type''=>''Int'',''percent_nbits''=>''Int'',''performance_options''=>''Int'',''rst''=>''Bool'',''use_almost_empty''=>''Bool'',''use_almost_full''=>''Bool'',''use_dcount''=>''Bool'',''use_percent_full_port''=>''Bool'',''xlcconfig''=>''String'',''block_type''=>''String''}';
      |   ptable_ = xlblockprep(get_param(tmp_gcb, 'MaskWSVariables'));
      |   try
      |     xlBlockMoveCallback(tmp_gcbh);
      |   catch 
      |      clear global xl_updateicon_recursion_guard;
      |   end;
      | catch
      |   global dbgsysgen;
      |   if(~isempty(dbgsysgen) && dbgsysgen)
      |     e = regexprep(lasterr, '\n', '\nError: ');
      |     disp(['Error: While running MaskInit code on block ' tmp_gcb ': ' e]);
      |     error(e);
      |   end
      | end
      settings: CopyFcn=xlBlockMoveCallback(gcbh);  DeleteFcn=xlDestroyGui(gcbh);  ModelCloseFcn=xlDestroyGui(gcbh);  PreSaveFcn=xlBlockPreSaveCallback(gcbh);  PostSaveFcn=xlBlockPostSaveCallback(gcbh);  DestroyFcn=xlDestroyGui(gcbh);  OpenFcn=xlOpenGui(gcbh, 'fifo_gui.xml', @fifoenablement, @fifoaction)  CloseFcn=xlDestroyGui(gcbh);  MoveFcn=xlBlockMoveCallback(gcbh);
      mask Help: eval('');xlDoc('-book','sysgen','-topic','FIFO');
      mask StyleString: edit,popup(Standard_FIFO|First_Word_Fall_Through),edit,popup(16|32|64|128|256|512|1K|2K|4K|8K|16K|32K|64K),edit,popup(1|2|3|4|5),edit,checkbox,edit,checkbox,edit,checkbox,edit,checkbox,edit,checkbox,edit,edit,checkbox,edit,edit,checkbox,edit,popup(Block RAM|Distributed RAM|Shift Register|Built-in FIFO),edit,checkbox,edit,edit,edit,edit,edit,edit,edit,edit,edit,edit,edit,edit,edit,edit,edit,edit,edit
      mask Display:
      | fprintf('','COMMENT: begin icon graphics');
      | patch([0 80 80 0 0 ],[0 0 114 114 0 ],[0.77 0.82 0.91 ]);
      | plot([0 80 80 0 0 ],[0 0 114 114 0 ]);
      | patch([15.525 31.42 42.42 53.42 64.42 42.42 26.525 15.525 ],[69.21 69.21 80.21 69.21 80.21 80.21 80.21 69.21 ],[1 1 1 ]);
      | patch([26.525 42.42 31.42 15.525 26.525 ],[58.21 58.21 69.21 69.21 58.21 ],[0.931 0.946 0.973 ]);
      | patch([15.525 31.42 42.42 26.525 15.525 ],[47.21 47.21 58.21 58.21 47.21 ],[1 1 1 ]);
      | patch([26.525 64.42 53.42 42.42 31.42 15.525 26.525 ],[36.21 36.21 47.21 36.21 47.21 47.21 36.21 ],[0.931 0.946 0.973 ]);
      | fprintf('','COMMENT: end icon graphics');
      | fprintf('','COMMENT: begin icon text');
      | color('black');port_label('input',1,'din');
      | color('black');port_label('input',2,'we');
      | color('black');port_label('input',3,'re');
      | color('black');port_label('output',1,'dout');
      | color('black');port_label('output',2,'empty');
      | color('black');port_label('output',3,'%full');
      | color('black');port_label('output',4,'full');
      | fprintf('','COMMENT: end icon text');
  "FIR Compiler 4.0 " : S-Function  LoadFcn=xlBlockLoadCallback(gcbh);  FunctionName=sysgen  Parameters=ptable_  EnableBusSupport=off  mask(Xilinx FIR Compiler 4.0 Block){coefficient_file=[1,2,3,4], coefficient_sets=1, filter_type=Single_Rate, rate_change_type=Integer, interpolation_rate=1, decimation_rate=1, zero_pack_factor=1, number_channels=1, ipcore_input_sample_period=1, filter_architecture=Systolic_Multiply_Accumulate, coefficient_reload=off, coefficient_structure=Inferred, coefficient_sign=Unsigned, quantization=Integer_Coefficients, coefficient_width=17, coefficient_fractional_bits=17, number_paths=1, output_rounding_mode=Full_Precision, output_width=36, allow_rounding_approximation=off, xl_use_area=off, xl_area=[0,0,0,0,0,0,0], optimization_goal=Area, rst=off, sclr_deterministic=on, en=off, has_nd=off, has_data_valid=off, usechan_in_adv=off, chan_in_adv=0, data_buffer_type=Automatic, coefficient_buffer_type=Automatic, input_buffer_type=Automatic, output_buffer_type=Automatic, preference_for_other_storage=Automatic, multi_column_support=Automatic, first_column_length=32, column_wrap_length=32, inter_column_pipe_length=4, passband_min=0.0, passband_max=0.5, stopband_min=0.5, stopband_max=1.0, filter_selection=1, has_sclr=true, sample_frequency=1.0, clock_frequency=1.0, data_sign=Signed, data_width=16, params_always_enabled={'usechan_in_adv','chan_in_adv'}, wrapper_available=true, ip_wrap_arbitrary_binary_point=true, ip_name=FIR Compiler, ip_version=4.0, dsptool_ready=true, ipcore_usecache=true, ipcore_useipmodelcache=true, ipcore_verbose=0, ipcore_xco_need_fpga_part=true, port_translation_map={ 'ce' => 'en', 'sclr' => 'rst', 'nd' => 'src_ce' }, run_core_at_system_period=true, ipcore_fpga_part=xlipgetpartsetting(gcb, {'virtex4', 'xc4vsx35', '-10', 'ff668'}), has_advanced_control=0, sggui_pos=-1,-1,-1,-1, block_type=fir_compiler_v4_0, block_version=, sg_icon_stat=95,142,-1,-1,white,blue,0,07734,right,,[ ],[ ], sg_mask_display=|, sg_list_contents=, sg_blockgui_xml=}
      mask sg_mask_display=|
      | fprintf('','COMMENT: begin icon graphics');
      | patch([0 95 95 0 0 ],[0 0 142 142 0 ],[0.77 0.82 0.91 ]);
      | plot([0 95 95 0 0 ],[0 0 142 142 0 ]);
      | patch([18.075 36.86 49.86 62.86 75.86 49.86 31.075 18.075 ],[85.43 85.43 98.43 85.43 98.43 98.43 98.43 85.43 ],[1 1 1 ]);
      | patch([31.075 49.86 36.86 18.075 31.075 ],[72.43 72.43 85.43 85.43 72.43 ],[0.931 0.946 0.973 ]);
      | patch([18.075 36.86 49.86 31.075 18.075 ],[59.43 59.43 72.43 72.43 59.43 ],[1 1 1 ]);
      | patch([31.075 75.86 62.86 49.86 36.86 18.075 31.075 ],[46.43 46.43 59.43 46.43 59.43 59.43 46.43 ],[0.931 0.946 0.973 ]);
      | fprintf('','COMMENT: end icon graphics');
      | fprintf('','COMMENT: begin icon text');
      | fprintf('','COMMENT: end icon text');
      mask prompts: coefficient_file "Coefficients"; coefficient_sets "Number of coefficient sets"; filter_type "Filter type"; rate_change_type "Rate change type"; interpolation_rate "Interpolation rate value"; decimation_rate "Decimation rate value"; zero_pack_factor "Zero pack factor"; number_channels "Number of channels"; ipcore_input_sample_period "Effective input sample period (clock_frequency / (sample_frequency * number_channels))"; filter_architecture "Filter architecture"; coefficient_reload "Use reloadable coefficients"; coefficient_structure "Coefficient structure"; coefficient_sign "Coefficient type"; coefficient_width "Coefficient width"; coefficient_fractional_bits "Coefficient fractional bits"; number_paths "Number of paths"; output_rounding_mode "Output rounding mode"; output_width "Output width"; allow_rounding_approximation "Allow rounding approximation"; xl_use_area "Define FPGA area for resource estimation"; xl_area "FPGA area [slices, FFs, BRAMs, LUTs, IOBs, emb. mults, TBUFs]"; optimization_goal "Optimization goal"; sclr_deterministic "Use deterministic rst behavior"; has_nd "nd"; has_data_valid "data_valid"; usechan_in_adv "Generate chan_in value in advance"; chan_in_adv "Number of samples"; data_buffer_type "Data buffer type"; coefficient_buffer_type "Coefficient buffer type"; input_buffer_type "Input buffer type"; output_buffer_type "Output buffer type"; preference_for_other_storage "Preference for other storage"; multi_column_support "Multi-column support"; first_column_length "First column length"; column_wrap_length "Column wrap length"; inter_column_pipe_length "Inter-column pipe length"; passband_min ""; passband_max ""; stopband_min ""; stopband_max ""; filter_selection ""; has_sclr ""; sample_frequency ""; clock_frequency ""; data_sign ""; data_width ""; params_always_enabled ""; wrapper_available ""; ip_wrap_arbitrary_binary_point ""; ip_name ""; ip_version ""; dsptool_ready ""; ipcore_usecache ""; ipcore_useipmodelcache ""; ipcore_verbose ""; ipcore_xco_need_fpga_part ""; port_translation_map ""; run_core_at_system_period ""; ipcore_fpga_part ""; has_advanced_control ""; sggui_pos ""; block_type ""; block_version ""; sg_icon_stat ""; sg_mask_display ""; sg_list_contents ""; sg_blockgui_xml ""
      mask help: Xilinx FIR Compiler 4.0
      mask init:
      | try
      |   tmp_gcb = gcb;
      |   tmp_gcbh = gcbh;
      |   if (strcmp('SysGenIndex',get_param(bdroot(tmp_gcbh),'tag')) && ~isempty(regexp(bdroot(tmp_gcb), '^xbs', 'once')))
      |     return;
      |   end;
      |   xlMungeMaskParams;
      |   block_config = 'sysgen_blockset:Removed_config';
      | 
      |   block_type='fir_compiler_v4_0';
      | nport = get_param(gcbh, 'ports');
      | nin = nport(1);
      | nout = nport(2);
      | 
      |   serialized_declarations = '{''allow_rounding_approximation''=>''Bool'',''chan_in_adv''=>''Int'',''clock_frequency''=>''Double'',''coefficient_buffer_type''=>''String'',''coefficient_file''=>''DoubleVector'',''coefficient_fractional_bits''=>''Int'',''coefficient_reload''=>''Bool'',''coefficient_sets''=>''Int'',''coefficient_sign''=>''String'',''coefficient_structure''=>''String'',''coefficient_width''=>''Int'',''column_wrap_length''=>''Int'',''data_buffer_type''=>''String'',''data_sign''=>''String'',''data_width''=>''Int'',''decimation_rate''=>''Int'',''dsptool_ready''=>''Bool'',''en''=>''Bool'',''filter_architecture''=>''String'',''filter_selection''=>''Int'',''filter_type''=>''String'',''first_column_length''=>''Int'',''has_data_valid''=>''Bool'',''has_nd''=>''Bool'',''has_sclr''=>''Bool'',''input_buffer_type''=>''String'',''inter_column_pipe_length''=>''Int'',''interpolation_rate''=>''Int'',''ip_name''=>''String'',''ip_version''=>''String'',''ip_wrap_arbitrary_binary_point''=>''Bool'',''ipcore_fpga_part''=>''StringVector'',''ipcore_input_sample_period''=>''Int'',''ipcore_usecache''=>''Bool'',''ipcore_useipmodelcache''=>''Bool'',''ipcore_verbose''=>''Bool'',''ipcore_xco_need_fpga_part''=>''Bool'',''multi_column_support''=>''String'',''number_channels''=>''Int'',''number_paths''=>''Int'',''optimization_goal''=>''String'',''output_buffer_type''=>''String'',''output_rounding_mode''=>''String'',''output_width''=>''Int'',''params_always_enabled''=>''String'',''passband_max''=>''Double'',''passband_min''=>''Double'',''port_translation_map''=>''String'',''preference_for_other_storage''=>''String'',''quantization''=>''String'',''rate_change_type''=>''String'',''rst''=>''Bool'',''run_core_at_system_period''=>''Bool'',''sample_frequency''=>''Double'',''sclr_deterministic''=>''Bool'',''stopband_max''=>''Double'',''stopband_min''=>''Double'',''usechan_in_adv''=>''Bool'',''wrapper_available''=>''Bool'',''xl_use_area''=>''Bool'',''zero_pack_factor''=>''Int'',''block_type''=>''String'',''nin''=>''Double'',''nout''=>''Double''}';
      |   ptable_ = xlblockprep(get_param(tmp_gcb, 'MaskWSVariables'));
      |   try
      |     xlBlockMoveCallback(tmp_gcbh);
      |   catch 
      |      clear global xl_updateicon_recursion_guard;
      |   end;
      | catch
      |   global dbgsysgen;
      |   if(~isempty(dbgsysgen) && dbgsysgen)
      |     e = regexprep(lasterr, '\n', '\nError: ');
      |     disp(['Error: While running MaskInit code on block ' tmp_gcb ': ' e]);
      |     error(e);
      |   end
      | end
      settings: CopyFcn=xlBlockMoveCallback(gcbh);  DeleteFcn=xlDestroyGui(gcbh);  ModelCloseFcn=xlDestroyGui(gcbh);  PreSaveFcn=xlBlockPreSaveCallback(gcbh);  PostSaveFcn=xlBlockPostSaveCallback(gcbh);  DestroyFcn=xlDestroyGui(gcbh);  OpenFcn=xlOpenGui(gcbh, 'fir_compiler_v4_0_gui.xml', @xlremovedenablement, -1)  CloseFcn=xlDestroyGui(gcbh);  MoveFcn=xlBlockMoveCallback(gcbh);
      mask Help: eval('');xlDoc('-book','sysgen','-topic','FIR_Compiler_4_0');
      mask StyleString: edit,edit,popup(Single_Rate|Interpolation|Decimation|Interpolated|Polyphase_Filter_Bank_Transmitter|Polyphase_Filter_Bank_Receiver),popup(Integer|Fixed_Fractional),edit,edit,edit,edit,edit,popup(Systolic_Multiply_Accumulate|Transpose_Multiply_Accumulate|Distributed_Arithmetic),checkbox,popup(Inferred|Non_Symmetric|Symmetric|Negative_Symmetric|Half_Band|Hilbert),popup(Signed|Unsigned),popup(Integer_Coefficients|Quantize_Only|Maximize_Dynamic_Range),edit,edit,edit,popup(Full_Precision|Truncate_LSBs|Non_Symmetric_Rounding_Down|Non_Symmetric_Rounding_Up|Symmetric_Rounding_to_Zero|Symmetric_Rounding_to_Infinity|Convergent_Rounding_to_Even|Convergent_Rounding_to_Odd),edit,checkbox,checkbox,edit,popup(Area|Speed),checkbox,checkbox,checkbox,checkbox,checkbox,checkbox,edit,popup(Automatic|Block|Distributed|Not_Applicable),popup(Automatic|Block|Distributed|Not_Applicable),popup(Automatic|Block|Distributed|Not_Applicable),popup(Automatic|Block|Distributed|Not_Applicable),popup(Automatic|Block|Distributed|Not_Applicable),popup(Disabled|Automatic|Custom),edit,edit,edit,edit,edit,edit,edit,edit,edit,edit,edit,edit,edit,edit,edit,edit,edit,edit,edit,edit,edit,edit,edit,edit,edit,edit,edit,edit,edit,edit,edit,edit,edit,edit
      mask Display:
      | fprintf('','COMMENT: begin icon graphics');
      | patch([0 95 95 0 0 ],[0 0 142 142 0 ],[0.77 0.82 0.91 ]);
      | plot([0 95 95 0 0 ],[0 0 142 142 0 ]);
      | patch([18.075 36.86 49.86 62.86 75.86 49.86 31.075 18.075 ],[85.43 85.43 98.43 85.43 98.43 98.43 98.43 85.43 ],[1 1 1 ]);
      | patch([31.075 49.86 36.86 18.075 31.075 ],[72.43 72.43 85.43 85.43 72.43 ],[0.931 0.946 0.973 ]);
      | patch([18.075 36.86 49.86 31.075 18.075 ],[59.43 59.43 72.43 72.43 59.43 ],[1 1 1 ]);
      | patch([31.075 75.86 62.86 49.86 36.86 18.075 31.075 ],[46.43 46.43 59.43 46.43 59.43 59.43 46.43 ],[0.931 0.946 0.973 ]);
      | fprintf('','COMMENT: end icon graphics');
      | fprintf('','COMMENT: begin icon text');
      | fprintf('','COMMENT: end icon text');
  "FIR Compiler 5.0 " : S-Function  LoadFcn=xlBlockLoadCallback(gcbh);  FunctionName=sysgen  Parameters=ptable_  EnableBusSupport=off  mask(Xilinx FIR Compiler 5.0 Block){coefficientvector=[6,0,-4,-3,5,6,-6,-13,7,44,64,44,7,-13,-6,6,5,-3,-4,0,6], coefficient_sets=1, filter_type=Single_Rate, rate_change_type=Integer, interpolation_rate=2, decimation_rate=1, zero_pack_factor=1, number_channels=1, ratespecification=Maximum_Possible, sampleperiod=1, hardwareoversamplingrate=1, filter_architecture=Systolic_Multiply_Accumulate, coefficient_reload=off, coefficient_structure=Inferred, coefficient_sign=Signed, quantization=Integer_Coefficients, coefficient_width=16, bestprecision=on, coefficient_fractional_bits=0, number_paths=1, output_rounding_mode=Full_Precision, output_width=24, allow_rounding_approximation=off, xl_use_area=off, xl_area=[0,0,0,0,0,0,0], optimization_goal=Area, has_sclr=off, has_data_valid=off, has_nd=off, has_ce=off, usechan_in_adv=off, chan_in_adv=0, data_buffer_type=Automatic, coefficient_buffer_type=Automatic, input_buffer_type=Automatic, output_buffer_type=Automatic, preference_for_other_storage=Automatic, multi_column_support=Disabled, columnconfig='1', inter_column_pipe_length=4, passband_min=0.0, passband_max=0.5, stopband_min=0.5, stopband_max=1.0, filter_selection=1, gui_behaviour=Sysgen, registered_output=true, data_sign=Signed, data_width=16, data_fractional_bits=0, wrapper_available=true, ip_wrap_arbitrary_binary_point=true, ip_name=FIR Compiler, ip_version=5.0, dsptool_ready=true, ipcore_usecache=true, ipcore_useipmodelcache=true, ipcore_xco_need_fpga_part=true, port_translation_map={ 'ce' => 'en', 'sclr' => 'rst' }, run_core_at_system_period=true, ipcore_fpga_part=xlipgetpartsetting(gcb, {'virtex4', 'xc4vsx35', '-10', 'ff668'}), structural_sim=false, has_advanced_control=0, sggui_pos=-1,-1,-1,-1, block_type=fir_compiler_v5_0, block_version=, sg_icon_stat=95,142,1,3,white,blue,0,671da946,right,,[ ],[ ], sg_mask_display=|, sg_list_contents=, sg_blockgui_xml=}
      mask sg_mask_display=|
      | fprintf('','COMMENT: begin icon graphics');
      | patch([0 95 95 0 0 ],[0 0 142 142 0 ],[0.77 0.82 0.91 ]);
      | plot([0 95 95 0 0 ],[0 0 142 142 0 ]);
      | patch([18.075 36.86 49.86 62.86 75.86 49.86 31.075 18.075 ],[85.43 85.43 98.43 85.43 98.43 98.43 98.43 85.43 ],[1 1 1 ]);
      | patch([31.075 49.86 36.86 18.075 31.075 ],[72.43 72.43 85.43 85.43 72.43 ],[0.931 0.946 0.973 ]);
      | patch([18.075 36.86 49.86 31.075 18.075 ],[59.43 59.43 72.43 72.43 59.43 ],[1 1 1 ]);
      | patch([31.075 75.86 62.86 49.86 36.86 18.075 31.075 ],[46.43 46.43 59.43 46.43 59.43 59.43 46.43 ],[0.931 0.946 0.973 ]);
      | fprintf('','COMMENT: end icon graphics');
      | fprintf('','COMMENT: begin icon text');
      | color('black');port_label('input',1,'din');
      | color('black');port_label('output',1,'dout');
      | color('black');port_label('output',2,'rfd');
      | color('black');port_label('output',3,'rdy');
      | fprintf('','COMMENT: end icon text');
      mask prompts: coefficientvector "Coefficient Vector :"; coefficient_sets "Number of Coefficient Sets :"; filter_type "Filter Type :"; rate_change_type "Rate Change Type :"; interpolation_rate "Interpolation Rate Value :"; decimation_rate "Decimation Rate Value :"; zero_pack_factor "Zero Pack Factor :"; number_channels "Number of Channels :"; ratespecification "Select format :"; sampleperiod "Sample period :"; hardwareoversamplingrate "Hardware Oversampling Rate :"; filter_architecture "Filter Architecture :"; coefficient_reload "Use Reloadable Coefficients"; coefficient_structure "Coefficient Structure :"; coefficient_sign "Coefficient Type :"; quantization "Quantization :"; coefficient_width "Coefficient Width :"; bestprecision "Best Precision Fraction Length"; coefficient_fractional_bits "Coefficient Fractional Bits :"; number_paths "Number of Paths :"; output_rounding_mode "Output Rounding Mode :"; output_width "Output Width :"; allow_rounding_approximation "Allow Rounding Approximation"; xl_use_area "Define FPGA area for resource estimation"; xl_area "FPGA area [slices, FFs, BRAMs, LUTs, IOBs, emb. mults, TBUFs]"; optimization_goal "Optimization Goal"; has_sclr "rst"; has_data_valid "data_valid"; has_nd "nd"; has_ce "ce"; usechan_in_adv "Generate CHAN_IN value in advance"; chan_in_adv "Number of samples:"; data_buffer_type "Data Buffer Type :"; coefficient_buffer_type "Coefficient Buffer Type :"; input_buffer_type "Input Buffer Type :"; output_buffer_type "Output Buffer Type :"; preference_for_other_storage "Preference for other storage :"; multi_column_support "Multi-Column Support :"; columnconfig "Column Configuration :"; inter_column_pipe_length "Inter-Column Pipe Length :"; passband_min ""; passband_max ""; stopband_min ""; stopband_max ""; filter_selection ""; gui_behaviour ""; registered_output ""; data_sign ""; data_width ""; data_fractional_bits ""; wrapper_available ""; ip_wrap_arbitrary_binary_point ""; ip_name ""; ip_version ""; dsptool_ready ""; ipcore_usecache ""; ipcore_useipmodelcache ""; ipcore_xco_need_fpga_part ""; port_translation_map ""; run_core_at_system_period ""; ipcore_fpga_part ""; structural_sim ""; has_advanced_control ""; sggui_pos ""; block_type ""; block_version ""; sg_icon_stat ""; sg_mask_display ""; sg_list_contents ""; sg_blockgui_xml ""
      mask help: Xilinx FIR Compiler 5.0
      mask init:
      | try
      |   tmp_gcb = gcb;
      |   tmp_gcbh = gcbh;
      |   if (strcmp('SysGenIndex',get_param(bdroot(tmp_gcbh),'tag')) && ~isempty(regexp(bdroot(tmp_gcb), '^xbs', 'once')))
      |     return;
      |   end;
      |   xlMungeMaskParams;
      |   block_config = 'sysgen:coregenimport_config';
      | 
      |   block_type='fir_compiler_v5_0';
      | 
      |   serialized_declarations = '{''allow_rounding_approximation''=>''Bool'',''bestprecision''=>''Bool'',''chan_in_adv''=>''Int'',''coefficient_buffer_type''=>''String'',''coefficient_fractional_bits''=>''Int'',''coefficient_reload''=>''Bool'',''coefficient_sets''=>''Int'',''coefficient_sign''=>''String'',''coefficient_structure''=>''String'',''coefficient_width''=>''Int'',''coefficientvector''=>''DoubleVector'',''columnconfig''=>''String'',''data_buffer_type''=>''String'',''data_fractional_bits''=>''Int'',''data_sign''=>''String'',''data_width''=>''Int'',''decimation_rate''=>''Int'',''dsptool_ready''=>''Bool'',''filter_architecture''=>''String'',''filter_selection''=>''Int'',''filter_type''=>''String'',''gui_behaviour''=>''String'',''hardwareoversamplingrate''=>''Int'',''has_ce''=>''Bool'',''has_data_valid''=>''Bool'',''has_nd''=>''Bool'',''has_sclr''=>''Bool'',''input_buffer_type''=>''String'',''inter_column_pipe_length''=>''Int'',''interpolation_rate''=>''Int'',''ip_name''=>''String'',''ip_version''=>''String'',''ip_wrap_arbitrary_binary_point''=>''Bool'',''ipcore_fpga_part''=>''StringVector'',''ipcore_usecache''=>''Bool'',''ipcore_useipmodelcache''=>''Bool'',''ipcore_xco_need_fpga_part''=>''Bool'',''multi_column_support''=>''String'',''number_channels''=>''Int'',''number_paths''=>''Int'',''optimization_goal''=>''String'',''output_buffer_type''=>''String'',''output_rounding_mode''=>''String'',''output_width''=>''Int'',''passband_max''=>''Double'',''passband_min''=>''Double'',''port_translation_map''=>''String'',''preference_for_other_storage''=>''String'',''quantization''=>''String'',''rate_change_type''=>''String'',''ratespecification''=>''String'',''registered_output''=>''Bool'',''run_core_at_system_period''=>''Bool'',''sampleperiod''=>''Int'',''stopband_max''=>''Double'',''stopband_min''=>''Double'',''structural_sim''=>''Bool'',''usechan_in_adv''=>''Bool'',''wrapper_available''=>''Bool'',''xl_use_area''=>''Bool'',''zero_pack_factor''=>''Int'',''block_type''=>''String''}';
      |   ptable_ = xlblockprep(get_param(tmp_gcb, 'MaskWSVariables'));
      |   try
      |     xlBlockMoveCallback(tmp_gcbh);
      |   catch 
      |      clear global xl_updateicon_recursion_guard;
      |   end;
      | catch
      |   global dbgsysgen;
      |   if(~isempty(dbgsysgen) && dbgsysgen)
      |     e = regexprep(lasterr, '\n', '\nError: ');
      |     disp(['Error: While running MaskInit code on block ' tmp_gcb ': ' e]);
      |     error(e);
      |   end
      | end
      settings: CopyFcn=xlBlockMoveCallback(gcbh);  DeleteFcn=xlDestroyGui(gcbh);  ModelCloseFcn=xlDestroyGui(gcbh);  PreSaveFcn=xlBlockPreSaveCallback(gcbh);  PostSaveFcn=xlBlockPostSaveCallback(gcbh);  DestroyFcn=xlDestroyGui(gcbh);  OpenFcn=xlOpenGui(gcbh, 'fir_compiler_v5_0_gui.xml', @xlipmagiccallback_pass_evaluate_params, @fir_compiler_v5_0_action)  CloseFcn=xlDestroyGui(gcbh);  MoveFcn=xlBlockMoveCallback(gcbh);
      mask Help: eval('');xlDoc('-book','sysgen','-topic','FIR_Compiler_5_0');
      mask StyleString: edit,edit,popup(Single_Rate|Interpolation|Decimation|Interpolated|Polyphase_Filter_Bank_Receiver|Polyphase_Filter_Bank_Transmitter),popup(Integer|Fixed_Fractional),edit,edit,edit,edit,popup(Maximum_Possible|Sample_Period|Hardware_Oversampling_Rate),edit,edit,popup(Systolic_Multiply_Accumulate|Transpose_Multiply_Accumulate|Distributed_Arithmetic),checkbox,popup(Inferred|Non_Symmetric|Symmetric|Negative_Symmetric|Half_Band|Hilbert),popup(Signed|Unsigned),popup(Integer_Coefficients|Quantize_Only|Maximize_Dynamic_Range),edit,checkbox,edit,edit,popup(Full_Precision|Truncate_LSBs|Non_Symmetric_Rounding_Down|Non_Symmetric_Rounding_Up|Symmetric_Rounding_to_Zero|Symmetric_Rounding_to_Infinity|Convergent_Rounding_to_Even|Convergent_Rounding_to_Odd),edit,checkbox,checkbox,edit,popup(Area|Speed),checkbox,checkbox,checkbox,checkbox,checkbox,edit,popup(Automatic|Block|Distributed|Not_Applicable),popup(Automatic|Block|Distributed|Not_Applicable),popup(Automatic|Block|Distributed|Not_Applicable),popup(Automatic|Block|Distributed|Not_Applicable),popup(Automatic|Block|Distributed|Not_Applicable),popup(Disabled|Automatic|Custom),edit,edit,edit,edit,edit,edit,edit,edit,edit,edit,edit,edit,edit,edit,edit,edit,edit,edit,edit,edit,edit,edit,edit,edit,edit,edit,edit,edit,edit,edit,edit,edit
      mask Display:
      | fprintf('','COMMENT: begin icon graphics');
      | patch([0 95 95 0 0 ],[0 0 142 142 0 ],[0.77 0.82 0.91 ]);
      | plot([0 95 95 0 0 ],[0 0 142 142 0 ]);
      | patch([18.075 36.86 49.86 62.86 75.86 49.86 31.075 18.075 ],[85.43 85.43 98.43 85.43 98.43 98.43 98.43 85.43 ],[1 1 1 ]);
      | patch([31.075 49.86 36.86 18.075 31.075 ],[72.43 72.43 85.43 85.43 72.43 ],[0.931 0.946 0.973 ]);
      | patch([18.075 36.86 49.86 31.075 18.075 ],[59.43 59.43 72.43 72.43 59.43 ],[1 1 1 ]);
      | patch([31.075 75.86 62.86 49.86 36.86 18.075 31.075 ],[46.43 46.43 59.43 46.43 59.43 59.43 46.43 ],[0.931 0.946 0.973 ]);
      | fprintf('','COMMENT: end icon graphics');
      | fprintf('','COMMENT: begin icon text');
      | color('black');port_label('input',1,'din');
      | color('black');port_label('output',1,'dout');
      | color('black');port_label('output',2,'rfd');
      | color('black');port_label('output',3,'rdy');
      | fprintf('','COMMENT: end icon text');
  "FIR Compiler 6.0 " : S-Function  LoadFcn=xlBlockLoadCallback(gcbh);  FunctionName=sysgen  Parameters=ptable_  EnableBusSupport=off  mask(Xilinx FIR Compiler 6.0 Block){coefficientvector=[6,0,-4,-3,5,6,-6,-13,7,44,64,44,7,-13,-6,6,5,-3,-4,0,6], coefficient_sets=1, filter_type=Single_Rate, interpolation_rate=1, decimation_rate=1, number_channels=1, infoedit=Maximum Possible : Maximizes oversampling rate. Abstracted input handshake (no s_data_tvalid) and automatic rate propagation.<br>Hardware Oversampling Rate : Specifies oversampling rate relative to the input sample period. Abstracted input handshake (no s_data_tvalid) and automatic rate propagation.<br>Sample Period : Specifies absolute oversampling rate. No input handshake abstraction (exposes s_data_tvalid) and no rate propagation., ratespecification=Maximum_Possible, sampleperiod=1, hardwareoversamplingrate=1, coefficient_reload=off, coefficient_sign=Signed, quantization=Integer_Coefficients, coefficient_width=16, bestprecision=on, coefficient_fractional_bits=0, coefficient_structure=Inferred, number_paths=1, output_rounding_mode=Full_Precision, output_width=24, xl_use_area=off, xl_area=[0,0,0,0,0,0,0], optimization_goal=Area, data_has_tlast=Not_Required, m_data_has_tready=off, s_data_has_tuser=Not_Required, m_data_has_tuser=Not_Required, s_config_sync_mode=On_Vector, s_config_method=Single, num_reload_slots=1, has_aclken=off, has_aresetn=off, multi_column_support=Disabled, columnconfig='1', inter_column_pipe_length=4, data_buffer_type=Automatic, coefficient_buffer_type=Automatic, input_buffer_type=Automatic, output_buffer_type=Automatic, preference_for_other_storage=Automatic, trim_axipin_name=on, passband_min=0.0, passband_max=0.5, stopband_min=0.5, stopband_max=1.0, filter_selection=1, gui_behaviour=Sysgen_GUI, data_sign=Signed, data_width=16, data_fractional_bits=0, wrapper_available=true, ip_wrap_arbitrary_binary_point=true, ip_name=FIR Compiler, ip_version=6.0, dsptool_ready=true, ipcore_usecache=true, ipcore_useipmodelcache=true, ipcore_xco_need_fpga_part=true, port_translation_map={ 'aclken' => 'en', 'aresetn' => 'rst' }, run_core_at_system_period=true, ipcore_fpga_part=xlipgetpartsetting(gcb, {'virtex6', 'xc6vlx75t', '-3', 'ff784'}), structural_sim=false, has_advanced_control=0, sggui_pos=-1,-1,-1,-1, block_type=fir_compiler_v6_0, block_version=, sg_icon_stat=240,206,1,3,white,blue,0,f63fefcf,right,,[2 ],[2 3 3 ], sg_mask_display=|, sg_list_contents=, sg_blockgui_xml=}
      mask sg_mask_display=|
      | fprintf('','COMMENT: begin icon graphics');
      | patch([0 0 4 4 ],[172 34 34 172 ],[5.466667e-001 5.800000e-001 6.400000e-001 ]);
      | patch([236 236 240 240 ],[197 149 149 197 ],[5.466667e-001 5.800000e-001 6.400000e-001 ]);
      | patch([236 236 240 240 ],[127 9 9 127 ],[3.233333e-001 3.400000e-001 3.700000e-001 ]);
      | patch([4 235 235 4 4 ],[0 0 206 206 0 ],[7.700000e-001 8.200000e-001 9.100000e-001 ]);
      | plot([4 235 235 4 4 ],[0 0 206 206 0 ]);
      |
      |
      | patch([55.475 97.38 126.38 155.38 184.38 126.38 84.475 55.475 ],[135.19 135.19 164.19 135.19 164.19 164.19 164.19 135.19 ],[1 1 1 ]);
      | patch([84.475 126.38 97.38 55.475 84.475 ],[106.19 106.19 135.19 135.19 106.19 ],[0.931 0.946 0.973 ]);
      | patch([55.475 97.38 126.38 84.475 55.475 ],[77.19 77.19 106.19 106.19 77.19 ],[1 1 1 ]);
      | patch([84.475 184.38 155.38 126.38 97.38 55.475 84.475 ],[48.19 48.19 77.19 48.19 77.19 77.19 48.19 ],[0.931 0.946 0.973 ]);
      | fprintf('','COMMENT: end icon graphics');
      | fprintf('','COMMENT: begin icon text');
      | color('black');port_label('input',1,'  data_tdata  ');
      | color('black');port_label('output',1,'  data_tready  ');
      | color('black');port_label('output',2,'  data_tvalid  ');
      | color('black');port_label('output',3,'  data_tdata  ');
      | fprintf('','COMMENT: end icon text');
      mask prompts: coefficientvector "Coefficient Vector :"; coefficient_sets "Number of Coefficient Sets :"; filter_type "Filter Type :"; interpolation_rate "Interpolation Rate Value :"; decimation_rate "Decimation Rate Value :"; number_channels "Number of Channels :"; infoedit ""; ratespecification "Select format :"; sampleperiod "Sample period :"; hardwareoversamplingrate "Hardware Oversampling Rate :"; coefficient_reload "Use Reloadable Coefficients"; coefficient_sign "Coefficient Type :"; quantization "Quantization :"; coefficient_width "Coefficient Width :"; bestprecision "Best Precision Fraction Length"; coefficient_fractional_bits "Coefficient Fractional Bits :"; coefficient_structure "Coefficient Structure :"; number_paths "Number of Paths :"; output_rounding_mode "Output Rounding Mode :"; output_width "Output Width :"; xl_use_area "Define FPGA area for resource estimation"; xl_area "FPGA area [slices, FFs, BRAMs, LUTs, IOBs, emb. mults, TBUFs]"; optimization_goal "Optimization Goal"; data_has_tlast "TLAST"; m_data_has_tready "Output TREADY"; s_data_has_tuser "Input :"; m_data_has_tuser "Output :"; s_config_sync_mode "Synchronization Mode :"; s_config_method "Configuration Method :"; num_reload_slots "Num reload slots"; has_aclken "ACLKEN"; has_aresetn "ARESETn"; multi_column_support "Multi-Column Support :"; columnconfig "Column Configuration :"; inter_column_pipe_length "Inter-Column Pipe Length :"; data_buffer_type "Data Buffer Type :"; coefficient_buffer_type "Coefficient Buffer Type :"; input_buffer_type "Input Buffer Type :"; output_buffer_type "Output Buffer Type :"; preference_for_other_storage "Preference for other storage :"; trim_axipin_name "Display shortened port names"; passband_min ""; passband_max ""; stopband_min ""; stopband_max ""; filter_selection ""; gui_behaviour ""; data_sign ""; data_width ""; data_fractional_bits ""; wrapper_available ""; ip_wrap_arbitrary_binary_point ""; ip_name ""; ip_version ""; dsptool_ready ""; ipcore_usecache ""; ipcore_useipmodelcache ""; ipcore_xco_need_fpga_part ""; port_translation_map ""; run_core_at_system_period ""; ipcore_fpga_part ""; structural_sim ""; has_advanced_control ""; sggui_pos ""; block_type ""; block_version ""; sg_icon_stat ""; sg_mask_display ""; sg_list_contents ""; sg_blockgui_xml ""
      mask help:
      | Maximum Possible : Maximizes oversampling rate. Abstracted input handshake (no s_data_tvalid) and automatic rate propagation.
      | Hardware Oversampling Rate : Specifies oversampling rate relative to the input sample period. Abstracted input handshake (no s_data_tvalid) and automatic rate propagation.
      | Sample Period : Specifies absolute oversampling rate. No input handshake abstraction (exposes s_data_tvalid) and no rate propagation.
      mask init:
      | try
      |   tmp_gcb = gcb;
      |   tmp_gcbh = gcbh;
      |   if (strcmp('SysGenIndex',get_param(bdroot(tmp_gcbh),'tag')) && ~isempty(regexp(bdroot(tmp_gcb), '^xbs', 'once')))
      |     return;
      |   end;
      |   xlMungeMaskParams;
      |   block_config = 'sysgen:coregenimport_config';
      | 
      |   block_type='fir_compiler_v6_0';
      | 
      |   serialized_declarations = '{''bestprecision''=>''Bool'',''coefficient_buffer_type''=>''String'',''coefficient_fractional_bits''=>''Int'',''coefficient_reload''=>''Bool'',''coefficient_sets''=>''Int'',''coefficient_sign''=>''String'',''coefficient_structure''=>''String'',''coefficient_width''=>''Int'',''coefficientvector''=>''DoubleVector'',''columnconfig''=>''String'',''data_buffer_type''=>''String'',''data_fractional_bits''=>''Int'',''data_has_tlast''=>''String'',''data_sign''=>''String'',''data_width''=>''Int'',''decimation_rate''=>''Int'',''dsptool_ready''=>''Bool'',''filter_selection''=>''Int'',''filter_type''=>''String'',''gui_behaviour''=>''String'',''hardwareoversamplingrate''=>''Int'',''has_aclken''=>''Bool'',''has_aresetn''=>''Bool'',''input_buffer_type''=>''String'',''inter_column_pipe_length''=>''Int'',''interpolation_rate''=>''Int'',''ip_name''=>''String'',''ip_version''=>''String'',''ip_wrap_arbitrary_binary_point''=>''Bool'',''ipcore_fpga_part''=>''StringVector'',''ipcore_usecache''=>''Bool'',''ipcore_useipmodelcache''=>''Bool'',''ipcore_xco_need_fpga_part''=>''Bool'',''m_data_has_tready''=>''Bool'',''m_data_has_tuser''=>''String'',''multi_column_support''=>''String'',''num_reload_slots''=>''Int'',''number_channels''=>''Int'',''number_paths''=>''Int'',''optimization_goal''=>''String'',''output_buffer_type''=>''String'',''output_rounding_mode''=>''String'',''output_width''=>''Int'',''passband_max''=>''Double'',''passband_min''=>''Double'',''port_translation_map''=>''String'',''preference_for_other_storage''=>''String'',''quantization''=>''String'',''ratespecification''=>''String'',''run_core_at_system_period''=>''Bool'',''s_config_method''=>''String'',''s_config_sync_mode''=>''String'',''s_data_has_tuser''=>''String'',''sampleperiod''=>''Int'',''stopband_max''=>''Double'',''stopband_min''=>''Double'',''structural_sim''=>''Bool'',''trim_axipin_name''=>''Int'',''wrapper_available''=>''Bool'',''xl_use_area''=>''Bool'',''block_type''=>''String''}';
      |   ptable_ = xlblockprep(get_param(tmp_gcb, 'MaskWSVariables'));
      |   try
      |     xlBlockMoveCallback(tmp_gcbh);
      |   catch 
      |      clear global xl_updateicon_recursion_guard;
      |   end;
      | catch
      |   global dbgsysgen;
      |   if(~isempty(dbgsysgen) && dbgsysgen)
      |     e = regexprep(lasterr, '\n', '\nError: ');
      |     disp(['Error: While running MaskInit code on block ' tmp_gcb ': ' e]);
      |     error(e);
      |   end
      | end
      settings: CopyFcn=xlBlockMoveCallback(gcbh);  DeleteFcn=xlDestroyGui(gcbh);  ModelCloseFcn=xlDestroyGui(gcbh);  PreSaveFcn=xlBlockPreSaveCallback(gcbh);  PostSaveFcn=xlBlockPostSaveCallback(gcbh);  DestroyFcn=xlDestroyGui(gcbh);  OpenFcn=xlOpenGui(gcbh, 'fir_compiler_v6_0_gui.xml', @xlipmagiccallback_pass_evaluate_params, @xlipmagicaction)  CloseFcn=xlDestroyGui(gcbh);  MoveFcn=xlBlockMoveCallback(gcbh);
      mask Help: eval('');xlDoc('-book','sysgen','-topic','FIR_Compiler_6_0');
      mask StyleString: edit,edit,popup(Single_Rate|Interpolation|Decimation),edit,edit,edit,edit,popup(Maximum_Possible|Sample_Period|Hardware_Oversampling_Rate),edit,edit,checkbox,popup(Signed|Unsigned),popup(Integer_Coefficients|Quantize_Only|Maximize_Dynamic_Range),edit,checkbox,edit,popup(Inferred|Non_Symmetric|Symmetric|Negative_Symmetric|Half_Band),edit,popup(Full_Precision|Truncate_LSBs|Non_Symmetric_Rounding_Down|Non_Symmetric_Rounding_Up|Symmetric_Rounding_to_Zero|Symmetric_Rounding_to_Infinity|Convergent_Rounding_to_Even|Convergent_Rounding_to_Odd),edit,checkbox,edit,popup(Area|Speed),popup(Not_Required|Vector_Framing|Packet_Framing),checkbox,popup(Not_Required|User_Field|Chan_ID_Field|User_and_Chan_ID_Field),popup(Not_Required|User_Field|Chan_ID_Field|User_and_Chan_ID_Field),popup(On_Vector|On_Packet),popup(Single|By_Channel),edit,checkbox,checkbox,popup(Disabled|Automatic|Custom),edit,edit,popup(Automatic|Block|Distributed|Not_Applicable),popup(Automatic|Block|Distributed|Not_Applicable),popup(Automatic|Block|Distributed|Not_Applicable),popup(Automatic|Block|Distributed|Not_Applicable),popup(Automatic|Block|Distributed|Not_Applicable),checkbox,edit,edit,edit,edit,edit,edit,edit,edit,edit,edit,edit,edit,edit,edit,edit,edit,edit,edit,edit,edit,edit,edit,edit,edit,edit,edit,edit,edit,edit
      mask Display:
      | fprintf('','COMMENT: begin icon graphics');
      | patch([0 0 4 4 ],[172 34 34 172 ],[5.466667e-001 5.800000e-001 6.400000e-001 ]);
      | patch([236 236 240 240 ],[197 149 149 197 ],[5.466667e-001 5.800000e-001 6.400000e-001 ]);
      | patch([236 236 240 240 ],[127 9 9 127 ],[3.233333e-001 3.400000e-001 3.700000e-001 ]);
      | patch([4 235 235 4 4 ],[0 0 206 206 0 ],[7.700000e-001 8.200000e-001 9.100000e-001 ]);
      | plot([4 235 235 4 4 ],[0 0 206 206 0 ]);
      | 
      | 
      | patch([55.475 97.38 126.38 155.38 184.38 126.38 84.475 55.475 ],[135.19 135.19 164.19 135.19 164.19 164.19 164.19 135.19 ],[1 1 1 ]);
      | patch([84.475 126.38 97.38 55.475 84.475 ],[106.19 106.19 135.19 135.19 106.19 ],[0.931 0.946 0.973 ]);
      | patch([55.475 97.38 126.38 84.475 55.475 ],[77.19 77.19 106.19 106.19 77.19 ],[1 1 1 ]);
      | patch([84.475 184.38 155.38 126.38 97.38 55.475 84.475 ],[48.19 48.19 77.19 48.19 77.19 77.19 48.19 ],[0.931 0.946 0.973 ]);
      | fprintf('','COMMENT: end icon graphics');
      | fprintf('','COMMENT: begin icon text');
      | color('black');port_label('input',1,'  data_tdata  ');
      | color('black');port_label('output',1,'  data_tready  ');
      | color('black');port_label('output',2,'  data_tvalid  ');
      | color('black');port_label('output',3,'  data_tdata  ');
      | fprintf('','COMMENT: end icon text');
  "FIR Compiler 6.1 " : S-Function  LoadFcn=xlBlockLoadCallback(gcbh);  FunctionName=sysgen  Parameters=ptable_  EnableBusSupport=off  mask(Xilinx FIR Compiler 6.1 Block){coefficientvector=[6,0,-4,-3,5,6,-6,-13,7,44,64,44,7,-13,-6,6,5,-3,-4,0,6], coefficient_sets=1, filter_type=Single_Rate, rate_change_type=Integer, interpolation_rate=1, decimation_rate=1, number_channels=1, infoedit=Maximum Possible : Maximizes oversampling rate. Abstracted input handshake (no s_data_tvalid) and automatic rate propagation.<br>Hardware Oversampling Rate : Specifies oversampling rate relative to the input sample period. Abstracted input handshake (no s_data_tvalid) and automatic rate propagation.<br>Sample Period : Specifies absolute oversampling rate. No input handshake abstraction (exposes s_data_tvalid) and no rate propagation., ratespecification=Maximum_Possible, sampleperiod=1, hardwareoversamplingrate=1, coefficient_reload=off, coefficient_sign=Signed, quantization=Integer_Coefficients, coefficient_width=16, bestprecision=on, coefficient_fractional_bits=0, coefficient_structure=Inferred, number_paths=1, output_rounding_mode=Full_Precision, output_width=24, xl_use_area=off, xl_area=[0,0,0,0,0,0,0], optimization_goal=Area, data_has_tlast=Not_Required, m_data_has_tready=off, s_data_has_tuser=Not_Required, m_data_has_tuser=Not_Required, s_config_sync_mode=On_Vector, s_config_method=Single, num_reload_slots=1, has_aclken=off, has_aresetn=off, multi_column_support=Disabled, columnconfig='1', inter_column_pipe_length=4, data_buffer_type=Automatic, coefficient_buffer_type=Automatic, input_buffer_type=Automatic, output_buffer_type=Automatic, preference_for_other_storage=Automatic, trim_axipin_name=on, passband_min=0.0, passband_max=0.5, stopband_min=0.5, stopband_max=1.0, filter_selection=1, gui_behaviour=Sysgen_GUI, data_sign=Signed, data_width=16, data_fractional_bits=0, wrapper_available=true, ip_wrap_arbitrary_binary_point=true, ip_name=FIR Compiler, ip_version=6.1, dsptool_ready=true, ipcore_usecache=true, ipcore_useipmodelcache=true, ipcore_xco_need_fpga_part=true, port_translation_map={ 'aclken' => 'en', 'aresetn' => 'rst' }, run_core_at_system_period=true, ipcore_fpga_part=xlipgetpartsetting(gcb, {'virtex6', 'xc6vlx75t', '-3', 'ff784'}), structural_sim=false, has_advanced_control=0, sggui_pos=-1,-1,-1,-1, block_type=fir_compiler_v6_1, block_version=, sg_icon_stat=240,206,1,3,white,blue,0,f63fefcf,right,,[2 ],[2 3 3 ], sg_mask_display=|, sg_list_contents=, sg_blockgui_xml=}
      mask sg_mask_display=|
      | fprintf('','COMMENT: begin icon graphics');
      | patch([0 0 4 4 ],[172 34 34 172 ],[5.466667e-001 5.800000e-001 6.400000e-001 ]);
      | patch([236 236 240 240 ],[197 149 149 197 ],[5.466667e-001 5.800000e-001 6.400000e-001 ]);
      | patch([236 236 240 240 ],[127 9 9 127 ],[3.233333e-001 3.400000e-001 3.700000e-001 ]);
      | patch([4 235 235 4 4 ],[0 0 206 206 0 ],[7.700000e-001 8.200000e-001 9.100000e-001 ]);
      | plot([4 235 235 4 4 ],[0 0 206 206 0 ]);
      |
      |
      | patch([55.475 97.38 126.38 155.38 184.38 126.38 84.475 55.475 ],[135.19 135.19 164.19 135.19 164.19 164.19 164.19 135.19 ],[1 1 1 ]);
      | patch([84.475 126.38 97.38 55.475 84.475 ],[106.19 106.19 135.19 135.19 106.19 ],[0.931 0.946 0.973 ]);
      | patch([55.475 97.38 126.38 84.475 55.475 ],[77.19 77.19 106.19 106.19 77.19 ],[1 1 1 ]);
      | patch([84.475 184.38 155.38 126.38 97.38 55.475 84.475 ],[48.19 48.19 77.19 48.19 77.19 77.19 48.19 ],[0.931 0.946 0.973 ]);
      | fprintf('','COMMENT: end icon graphics');
      | fprintf('','COMMENT: begin icon text');
      | color('black');port_label('input',1,'  data_tdata  ');
      | color('black');port_label('output',1,'  data_tready  ');
      | color('black');port_label('output',2,'  data_tvalid  ');
      | color('black');port_label('output',3,'  data_tdata  ');
      | fprintf('','COMMENT: end icon text');
      mask prompts: coefficientvector "Coefficient Vector :"; coefficient_sets "Number of Coefficient Sets :"; filter_type "Filter Type :"; rate_change_type "Rate Change Type :"; interpolation_rate "Interpolation Rate Value :"; decimation_rate "Decimation Rate Value :"; number_channels "Number of Channels :"; infoedit ""; ratespecification "Select format :"; sampleperiod "Sample period :"; hardwareoversamplingrate "Hardware Oversampling Rate :"; coefficient_reload "Use Reloadable Coefficients"; coefficient_sign "Coefficient Type :"; quantization "Quantization :"; coefficient_width "Coefficient Width :"; bestprecision "Best Precision Fraction Length"; coefficient_fractional_bits "Coefficient Fractional Bits :"; coefficient_structure "Coefficient Structure :"; number_paths "Number of Paths :"; output_rounding_mode "Output Rounding Mode :"; output_width "Output Width :"; xl_use_area "Define FPGA area for resource estimation"; xl_area "FPGA area [slices, FFs, BRAMs, LUTs, IOBs, emb. mults, TBUFs]"; optimization_goal "Optimization Goal"; data_has_tlast "TLAST"; m_data_has_tready "Output TREADY"; s_data_has_tuser "Input :"; m_data_has_tuser "Output :"; s_config_sync_mode "Synchronization Mode :"; s_config_method "Configuration Method :"; num_reload_slots "Num reload slots"; has_aclken "ACLKEN"; has_aresetn "ARESETn"; multi_column_support "Multi-Column Support :"; columnconfig "Column Configuration :"; inter_column_pipe_length "Inter-Column Pipe Length :"; data_buffer_type "Data Buffer Type :"; coefficient_buffer_type "Coefficient Buffer Type :"; input_buffer_type "Input Buffer Type :"; output_buffer_type "Output Buffer Type :"; preference_for_other_storage "Preference for other storage :"; trim_axipin_name "Display shortened port names"; passband_min ""; passband_max ""; stopband_min ""; stopband_max ""; filter_selection ""; gui_behaviour ""; data_sign ""; data_width ""; data_fractional_bits ""; wrapper_available ""; ip_wrap_arbitrary_binary_point ""; ip_name ""; ip_version ""; dsptool_ready ""; ipcore_usecache ""; ipcore_useipmodelcache ""; ipcore_xco_need_fpga_part ""; port_translation_map ""; run_core_at_system_period ""; ipcore_fpga_part ""; structural_sim ""; has_advanced_control ""; sggui_pos ""; block_type ""; block_version ""; sg_icon_stat ""; sg_mask_display ""; sg_list_contents ""; sg_blockgui_xml ""
      mask help:
      | Maximum Possible : Maximizes oversampling rate. Abstracted input handshake (no s_data_tvalid) and automatic rate propagation.
      | Hardware Oversampling Rate : Specifies oversampling rate relative to the input sample period. Abstracted input handshake (no s_data_tvalid) and automatic rate propagation.
      | Sample Period : Specifies absolute oversampling rate. No input handshake abstraction (exposes s_data_tvalid) and no rate propagation.
      mask init:
      | try
      |   tmp_gcb = gcb;
      |   tmp_gcbh = gcbh;
      |   if (strcmp('SysGenIndex',get_param(bdroot(tmp_gcbh),'tag')) && ~isempty(regexp(bdroot(tmp_gcb), '^xbs', 'once')))
      |     return;
      |   end;
      |   xlMungeMaskParams;
      |   block_config = 'sysgen:coregenimport_config';
      | 
      |   block_type='fir_compiler_v6_1';
      | 
      |   serialized_declarations = '{''bestprecision''=>''Bool'',''coefficient_buffer_type''=>''String'',''coefficient_fractional_bits''=>''Int'',''coefficient_reload''=>''Bool'',''coefficient_sets''=>''Int'',''coefficient_sign''=>''String'',''coefficient_structure''=>''String'',''coefficient_width''=>''Int'',''coefficientvector''=>''DoubleVector'',''columnconfig''=>''String'',''data_buffer_type''=>''String'',''data_fractional_bits''=>''Int'',''data_has_tlast''=>''String'',''data_sign''=>''String'',''data_width''=>''Int'',''decimation_rate''=>''Int'',''dsptool_ready''=>''Bool'',''filter_selection''=>''Int'',''filter_type''=>''String'',''gui_behaviour''=>''String'',''hardwareoversamplingrate''=>''Int'',''has_aclken''=>''Bool'',''has_aresetn''=>''Bool'',''input_buffer_type''=>''String'',''inter_column_pipe_length''=>''Int'',''interpolation_rate''=>''Int'',''ip_name''=>''String'',''ip_version''=>''String'',''ip_wrap_arbitrary_binary_point''=>''Bool'',''ipcore_fpga_part''=>''StringVector'',''ipcore_usecache''=>''Bool'',''ipcore_useipmodelcache''=>''Bool'',''ipcore_xco_need_fpga_part''=>''Bool'',''m_data_has_tready''=>''Bool'',''m_data_has_tuser''=>''String'',''multi_column_support''=>''String'',''num_reload_slots''=>''Int'',''number_channels''=>''Int'',''number_paths''=>''Int'',''optimization_goal''=>''String'',''output_buffer_type''=>''String'',''output_rounding_mode''=>''String'',''output_width''=>''Int'',''passband_max''=>''Double'',''passband_min''=>''Double'',''port_translation_map''=>''String'',''preference_for_other_storage''=>''String'',''quantization''=>''String'',''rate_change_type''=>''String'',''ratespecification''=>''String'',''run_core_at_system_period''=>''Bool'',''s_config_method''=>''String'',''s_config_sync_mode''=>''String'',''s_data_has_tuser''=>''String'',''sampleperiod''=>''Int'',''stopband_max''=>''Double'',''stopband_min''=>''Double'',''structural_sim''=>''Bool'',''trim_axipin_name''=>''Int'',''wrapper_available''=>''Bool'',''xl_use_area''=>''Bool'',''block_type''=>''String''}';
      |   ptable_ = xlblockprep(get_param(tmp_gcb, 'MaskWSVariables'));
      |   try
      |     xlBlockMoveCallback(tmp_gcbh);
      |   catch 
      |      clear global xl_updateicon_recursion_guard;
      |   end;
      | catch
      |   global dbgsysgen;
      |   if(~isempty(dbgsysgen) && dbgsysgen)
      |     e = regexprep(lasterr, '\n', '\nError: ');
      |     disp(['Error: While running MaskInit code on block ' tmp_gcb ': ' e]);
      |     error(e);
      |   end
      | end
      settings: CopyFcn=xlBlockMoveCallback(gcbh);  DeleteFcn=xlDestroyGui(gcbh);  ModelCloseFcn=xlDestroyGui(gcbh);  PreSaveFcn=xlBlockPreSaveCallback(gcbh);  PostSaveFcn=xlBlockPostSaveCallback(gcbh);  DestroyFcn=xlDestroyGui(gcbh);  OpenFcn=xlOpenGui(gcbh, 'fir_compiler_v6_1_gui.xml', @xlipmagiccallback_pass_evaluate_params, -1)  CloseFcn=xlDestroyGui(gcbh);  MoveFcn=xlBlockMoveCallback(gcbh);
      mask Help: eval('');xlDoc('-book','sysgen','-topic','FIR_Compiler_6_1');
      mask StyleString: edit,edit,popup(Single_Rate|Interpolation|Decimation),popup(Integer|Fixed_Fractional),edit,edit,edit,edit,popup(Maximum_Possible|Sample_Period|Hardware_Oversampling_Rate),edit,edit,checkbox,popup(Signed|Unsigned),popup(Integer_Coefficients|Quantize_Only|Maximize_Dynamic_Range),edit,checkbox,edit,popup(Inferred|Non_Symmetric|Symmetric|Negative_Symmetric|Half_Band),edit,popup(Full_Precision|Truncate_LSBs|Non_Symmetric_Rounding_Down|Non_Symmetric_Rounding_Up|Symmetric_Rounding_to_Zero|Symmetric_Rounding_to_Infinity|Convergent_Rounding_to_Even|Convergent_Rounding_to_Odd),edit,checkbox,edit,popup(Area|Speed),popup(Not_Required|Vector_Framing|Packet_Framing),checkbox,popup(Not_Required|User_Field|Chan_ID_Field|User_and_Chan_ID_Field),popup(Not_Required|User_Field|Chan_ID_Field|User_and_Chan_ID_Field),popup(On_Vector|On_Packet),popup(Single|By_Channel),edit,checkbox,checkbox,popup(Disabled|Automatic|Custom),edit,edit,popup(Automatic|Block|Distributed|Not_Applicable),popup(Automatic|Block|Distributed|Not_Applicable),popup(Automatic|Block|Distributed|Not_Applicable),popup(Automatic|Block|Distributed|Not_Applicable),popup(Automatic|Block|Distributed|Not_Applicable),checkbox,edit,edit,edit,edit,edit,edit,edit,edit,edit,edit,edit,edit,edit,edit,edit,edit,edit,edit,edit,edit,edit,edit,edit,edit,edit,edit,edit,edit,edit
      mask Display:
      | fprintf('','COMMENT: begin icon graphics');
      | patch([0 0 4 4 ],[172 34 34 172 ],[5.466667e-001 5.800000e-001 6.400000e-001 ]);
      | patch([236 236 240 240 ],[197 149 149 197 ],[5.466667e-001 5.800000e-001 6.400000e-001 ]);
      | patch([236 236 240 240 ],[127 9 9 127 ],[3.233333e-001 3.400000e-001 3.700000e-001 ]);
      | patch([4 235 235 4 4 ],[0 0 206 206 0 ],[7.700000e-001 8.200000e-001 9.100000e-001 ]);
      | plot([4 235 235 4 4 ],[0 0 206 206 0 ]);
      | 
      | 
      | patch([55.475 97.38 126.38 155.38 184.38 126.38 84.475 55.475 ],[135.19 135.19 164.19 135.19 164.19 164.19 164.19 135.19 ],[1 1 1 ]);
      | patch([84.475 126.38 97.38 55.475 84.475 ],[106.19 106.19 135.19 135.19 106.19 ],[0.931 0.946 0.973 ]);
      | patch([55.475 97.38 126.38 84.475 55.475 ],[77.19 77.19 106.19 106.19 77.19 ],[1 1 1 ]);
      | patch([84.475 184.38 155.38 126.38 97.38 55.475 84.475 ],[48.19 48.19 77.19 48.19 77.19 77.19 48.19 ],[0.931 0.946 0.973 ]);
      | fprintf('','COMMENT: end icon graphics');
      | fprintf('','COMMENT: begin icon text');
      | color('black');port_label('input',1,'  data_tdata  ');
      | color('black');port_label('output',1,'  data_tready  ');
      | color('black');port_label('output',2,'  data_tvalid  ');
      | color('black');port_label('output',3,'  data_tdata  ');
      | fprintf('','COMMENT: end icon text');
  "FIR Compiler 6.2 " : S-Function  LoadFcn=xlBlockLoadCallback(gcbh);  FunctionName=sysgen  Parameters=ptable_  EnableBusSupport=off  mask(Xilinx FIR Compiler 6.2 Block){coefficientvector=[6,0,-4,-3,5,6,-6,-13,7,44,64,44,7,-13,-6,6,5,-3,-4,0,6], coefficient_sets=1, filter_type=Single_Rate, rate_change_type=Integer, interpolation_rate=1, decimation_rate=1, number_channels=1, infoedit=Maximum Possible : Maximizes oversampling rate. Abstracted input handshake (no s_data_tvalid) and automatic rate propagation.<br>Hardware Oversampling Rate : Specifies oversampling rate relative to the input sample period. Abstracted input handshake (no s_data_tvalid) and automatic rate propagation.<br>Sample Period : Specifies absolute oversampling rate. No input handshake abstraction (exposes s_data_tvalid) and no rate propagation., ratespecification=Maximum_Possible, sampleperiod=1, hardwareoversamplingrate=1, filter_architecture=Systolic_Multiply_Accumulate, coefficient_reload=off, coefficient_sign=Signed, quantization=Integer_Coefficients, coefficient_width=16, bestprecision=on, coefficient_fractional_bits=0, coefficient_structure=Inferred, number_paths=1, output_rounding_mode=Full_Precision, output_width=24, xl_use_area=off, xl_area=[0,0,0,0,0,0,0], optimization_goal=Area, data_has_tlast=Not_Required, m_data_has_tready=off, s_data_has_fifo=off, s_data_has_tuser=Not_Required, m_data_has_tuser=Not_Required, s_config_sync_mode=On_Vector, s_config_method=Single, num_reload_slots=1, has_aclken=off, has_aresetn=off, multi_column_support=Disabled, columnconfig='1', inter_column_pipe_length=4, data_buffer_type=Automatic, coefficient_buffer_type=Automatic, input_buffer_type=Automatic, output_buffer_type=Automatic, preference_for_other_storage=Automatic, trim_axipin_name=on, passband_min=0.0, passband_max=0.5, stopband_min=0.5, stopband_max=1.0, filter_selection=1, gui_behaviour=Sysgen_GUI, data_sign=Signed, data_width=16, data_fractional_bits=0, wrapper_available=true, ip_wrap_arbitrary_binary_point=true, ip_name=FIR Compiler, ip_version=6.2, dsptool_ready=true, ipcore_usecache=true, ipcore_useipmodelcache=true, ipcore_xco_need_fpga_part=true, port_translation_map={ 'aclken' => 'en', 'aresetn' => 'rst' }, run_core_at_system_period=true, ipcore_fpga_part=xlipgetpartsetting(gcb, {'virtex6', 'xc6vlx75t', '-3', 'ff784'}), structural_sim=false, has_advanced_control=0, sggui_pos=-1,-1,-1,-1, block_type=fir_compiler_v6_2, block_version=, sg_icon_stat=240,206,1,3,white,blue,0,f63fefcf,right,,[2 ],[2 3 3 ], sg_mask_display=|, sg_list_contents=, sg_blockgui_xml=}
      mask sg_mask_display=|
      | fprintf('','COMMENT: begin icon graphics');
      | patch([0 0 4 4 ],[172 34 34 172 ],[5.466667e-001 5.800000e-001 6.400000e-001 ]);
      | patch([236 236 240 240 ],[197 149 149 197 ],[5.466667e-001 5.800000e-001 6.400000e-001 ]);
      | patch([236 236 240 240 ],[127 9 9 127 ],[3.233333e-001 3.400000e-001 3.700000e-001 ]);
      | patch([4 235 235 4 4 ],[0 0 206 206 0 ],[7.700000e-001 8.200000e-001 9.100000e-001 ]);
      | plot([4 235 235 4 4 ],[0 0 206 206 0 ]);
      |
      |
      | patch([55.475 97.38 126.38 155.38 184.38 126.38 84.475 55.475 ],[135.19 135.19 164.19 135.19 164.19 164.19 164.19 135.19 ],[1 1 1 ]);
      | patch([84.475 126.38 97.38 55.475 84.475 ],[106.19 106.19 135.19 135.19 106.19 ],[0.931 0.946 0.973 ]);
      | patch([55.475 97.38 126.38 84.475 55.475 ],[77.19 77.19 106.19 106.19 77.19 ],[1 1 1 ]);
      | patch([84.475 184.38 155.38 126.38 97.38 55.475 84.475 ],[48.19 48.19 77.19 48.19 77.19 77.19 48.19 ],[0.931 0.946 0.973 ]);
      | fprintf('','COMMENT: end icon graphics');
      | fprintf('','COMMENT: begin icon text');
      | color('black');port_label('input',1,'  data_tdata  ');
      | color('black');port_label('output',1,'  data_tready  ');
      | color('black');port_label('output',2,'  data_tvalid  ');
      | color('black');port_label('output',3,'  data_tdata  ');
      | fprintf('','COMMENT: end icon text');
      mask prompts: coefficientvector "Coefficient Vector :"; coefficient_sets "Number of Coefficient Sets :"; filter_type "Filter Type :"; rate_change_type "Rate Change Type :"; interpolation_rate "Interpolation Rate Value :"; decimation_rate "Decimation Rate Value :"; number_channels "Number of Channels :"; infoedit ""; ratespecification "Select format :"; sampleperiod "Sample period :"; hardwareoversamplingrate "Hardware Oversampling Rate :"; filter_architecture "Filter Architecture :"; coefficient_reload "Use Reloadable Coefficients"; coefficient_sign "Coefficient Type :"; quantization "Quantization :"; coefficient_width "Coefficient Width :"; bestprecision "Best Precision Fraction Length"; coefficient_fractional_bits "Coefficient Fractional Bits :"; coefficient_structure "Coefficient Structure :"; number_paths "Number of Paths :"; output_rounding_mode "Output Rounding Mode :"; output_width "Output Width :"; xl_use_area "Define FPGA area for resource estimation"; xl_area "FPGA area [slices, FFs, BRAMs, LUTs, IOBs, emb. mults, TBUFs]"; optimization_goal "Optimization Goal"; data_has_tlast "TLAST"; m_data_has_tready "Output TREADY"; s_data_has_fifo "Input FIFO"; s_data_has_tuser "Input :"; m_data_has_tuser "Output :"; s_config_sync_mode "Synchronization Mode :"; s_config_method "Configuration Method :"; num_reload_slots "Num reload slots"; has_aclken "ACLKEN"; has_aresetn "ARESETn"; multi_column_support "Multi-Column Support :"; columnconfig "Column Configuration :"; inter_column_pipe_length "Inter-Column Pipe Length :"; data_buffer_type "Data Buffer Type :"; coefficient_buffer_type "Coefficient Buffer Type :"; input_buffer_type "Input Buffer Type :"; output_buffer_type "Output Buffer Type :"; preference_for_other_storage "Preference for other storage :"; trim_axipin_name "Display shortened port names"; passband_min ""; passband_max ""; stopband_min ""; stopband_max ""; filter_selection ""; gui_behaviour ""; data_sign ""; data_width ""; data_fractional_bits ""; wrapper_available ""; ip_wrap_arbitrary_binary_point ""; ip_name ""; ip_version ""; dsptool_ready ""; ipcore_usecache ""; ipcore_useipmodelcache ""; ipcore_xco_need_fpga_part ""; port_translation_map ""; run_core_at_system_period ""; ipcore_fpga_part ""; structural_sim ""; has_advanced_control ""; sggui_pos ""; block_type ""; block_version ""; sg_icon_stat ""; sg_mask_display ""; sg_list_contents ""; sg_blockgui_xml ""
      mask help:
      | Maximum Possible : Maximizes oversampling rate. Abstracted input handshake (no s_data_tvalid) and automatic rate propagation.
      | Hardware Oversampling Rate : Specifies oversampling rate relative to the input sample period. Abstracted input handshake (no s_data_tvalid) and automatic rate propagation.
      | Sample Period : Specifies absolute oversampling rate. No input handshake abstraction (exposes s_data_tvalid) and no rate propagation.
      mask init:
      | try
      |   tmp_gcb = gcb;
      |   tmp_gcbh = gcbh;
      |   if (strcmp('SysGenIndex',get_param(bdroot(tmp_gcbh),'tag')) && ~isempty(regexp(bdroot(tmp_gcb), '^xbs', 'once')))
      |     return;
      |   end;
      |   xlMungeMaskParams;
      |   block_config = 'sysgen:coregenimport_config';
      | 
      |   block_type='fir_compiler_v6_2';
      | 
      |   serialized_declarations = '{''bestprecision''=>''Bool'',''coefficient_buffer_type''=>''String'',''coefficient_fractional_bits''=>''Int'',''coefficient_reload''=>''Bool'',''coefficient_sets''=>''Int'',''coefficient_sign''=>''String'',''coefficient_structure''=>''String'',''coefficient_width''=>''Int'',''coefficientvector''=>''DoubleVector'',''columnconfig''=>''String'',''data_buffer_type''=>''String'',''data_fractional_bits''=>''Int'',''data_has_tlast''=>''String'',''data_sign''=>''String'',''data_width''=>''Int'',''decimation_rate''=>''Int'',''dsptool_ready''=>''Bool'',''filter_architecture''=>''String'',''filter_selection''=>''Int'',''filter_type''=>''String'',''gui_behaviour''=>''String'',''hardwareoversamplingrate''=>''Int'',''has_aclken''=>''Bool'',''has_aresetn''=>''Bool'',''input_buffer_type''=>''String'',''inter_column_pipe_length''=>''Int'',''interpolation_rate''=>''Int'',''ip_name''=>''String'',''ip_version''=>''String'',''ip_wrap_arbitrary_binary_point''=>''Bool'',''ipcore_fpga_part''=>''StringVector'',''ipcore_usecache''=>''Bool'',''ipcore_useipmodelcache''=>''Bool'',''ipcore_xco_need_fpga_part''=>''Bool'',''m_data_has_tready''=>''Bool'',''m_data_has_tuser''=>''String'',''multi_column_support''=>''String'',''num_reload_slots''=>''Int'',''number_channels''=>''Int'',''number_paths''=>''Int'',''optimization_goal''=>''String'',''output_buffer_type''=>''String'',''output_rounding_mode''=>''String'',''output_width''=>''Int'',''passband_max''=>''Double'',''passband_min''=>''Double'',''port_translation_map''=>''String'',''preference_for_other_storage''=>''String'',''quantization''=>''String'',''rate_change_type''=>''String'',''ratespecification''=>''String'',''run_core_at_system_period''=>''Bool'',''s_config_method''=>''String'',''s_config_sync_mode''=>''String'',''s_data_has_fifo''=>''Bool'',''s_data_has_tuser''=>''String'',''sampleperiod''=>''Int'',''stopband_max''=>''Double'',''stopband_min''=>''Double'',''structural_sim''=>''Bool'',''trim_axipin_name''=>''Int'',''wrapper_available''=>''Bool'',''xl_use_area''=>''Bool'',''block_type''=>''String''}';
      |   ptable_ = xlblockprep(get_param(tmp_gcb, 'MaskWSVariables'));
      |   try
      |     xlBlockMoveCallback(tmp_gcbh);
      |   catch 
      |      clear global xl_updateicon_recursion_guard;
      |   end;
      | catch
      |   global dbgsysgen;
      |   if(~isempty(dbgsysgen) && dbgsysgen)
      |     e = regexprep(lasterr, '\n', '\nError: ');
      |     disp(['Error: While running MaskInit code on block ' tmp_gcb ': ' e]);
      |     error(e);
      |   end
      | end
      settings: CopyFcn=xlBlockMoveCallback(gcbh);  DeleteFcn=xlDestroyGui(gcbh);  ModelCloseFcn=xlDestroyGui(gcbh);  PreSaveFcn=xlBlockPreSaveCallback(gcbh);  PostSaveFcn=xlBlockPostSaveCallback(gcbh);  DestroyFcn=xlDestroyGui(gcbh);  OpenFcn=xlOpenGui(gcbh, 'fir_compiler_v6_2_gui.xml', @xlipmagiccallback_pass_evaluate_params, @fir_compiler_v6_2_action)  CloseFcn=xlDestroyGui(gcbh);  MoveFcn=xlBlockMoveCallback(gcbh);
      mask Help: eval('');xlDoc('-book','sysgen','-topic','FIR_Compiler_6_2');
      mask StyleString: edit,edit,popup(Single_Rate|Interpolation|Decimation),popup(Integer|Fixed_Fractional),edit,edit,edit,edit,popup(Maximum_Possible|Sample_Period|Hardware_Oversampling_Rate),edit,edit,popup(Systolic_Multiply_Accumulate|Transpose_Multiply_Accumulate),checkbox,popup(Signed|Unsigned),popup(Integer_Coefficients|Quantize_Only|Maximize_Dynamic_Range),edit,checkbox,edit,popup(Inferred|Non_Symmetric|Symmetric|Negative_Symmetric|Half_Band),edit,popup(Full_Precision|Truncate_LSBs|Non_Symmetric_Rounding_Down|Non_Symmetric_Rounding_Up|Symmetric_Rounding_to_Zero|Symmetric_Rounding_to_Infinity|Convergent_Rounding_to_Even|Convergent_Rounding_to_Odd),edit,checkbox,edit,popup(Area|Speed),popup(Not_Required|Vector_Framing|Packet_Framing),checkbox,checkbox,popup(Not_Required|User_Field|Chan_ID_Field|User_and_Chan_ID_Field),popup(Not_Required|User_Field|Chan_ID_Field|User_and_Chan_ID_Field),popup(On_Vector|On_Packet),popup(Single|By_Channel),edit,checkbox,checkbox,popup(Disabled|Automatic|Custom),edit,edit,popup(Automatic|Block|Distributed|Not_Applicable),popup(Automatic|Block|Distributed|Not_Applicable),popup(Automatic|Block|Distributed|Not_Applicable),popup(Automatic|Block|Distributed|Not_Applicable),popup(Automatic|Block|Distributed|Not_Applicable),checkbox,edit,edit,edit,edit,edit,edit,edit,edit,edit,edit,edit,edit,edit,edit,edit,edit,edit,edit,edit,edit,edit,edit,edit,edit,edit,edit,edit,edit,edit
      mask Display:
      | fprintf('','COMMENT: begin icon graphics');
      | patch([0 0 4 4 ],[172 34 34 172 ],[5.466667e-001 5.800000e-001 6.400000e-001 ]);
      | patch([236 236 240 240 ],[197 149 149 197 ],[5.466667e-001 5.800000e-001 6.400000e-001 ]);
      | patch([236 236 240 240 ],[127 9 9 127 ],[3.233333e-001 3.400000e-001 3.700000e-001 ]);
      | patch([4 235 235 4 4 ],[0 0 206 206 0 ],[7.700000e-001 8.200000e-001 9.100000e-001 ]);
      | plot([4 235 235 4 4 ],[0 0 206 206 0 ]);
      | 
      | 
      | patch([55.475 97.38 126.38 155.38 184.38 126.38 84.475 55.475 ],[135.19 135.19 164.19 135.19 164.19 164.19 164.19 135.19 ],[1 1 1 ]);
      | patch([84.475 126.38 97.38 55.475 84.475 ],[106.19 106.19 135.19 135.19 106.19 ],[0.931 0.946 0.973 ]);
      | patch([55.475 97.38 126.38 84.475 55.475 ],[77.19 77.19 106.19 106.19 77.19 ],[1 1 1 ]);
      | patch([84.475 184.38 155.38 126.38 97.38 55.475 84.475 ],[48.19 48.19 77.19 48.19 77.19 77.19 48.19 ],[0.931 0.946 0.973 ]);
      | fprintf('','COMMENT: end icon graphics');
      | fprintf('','COMMENT: begin icon text');
      | color('black');port_label('input',1,'  data_tdata  ');
      | color('black');port_label('output',1,'  data_tready  ');
      | color('black');port_label('output',2,'  data_tvalid  ');
      | color('black');port_label('output',3,'  data_tdata  ');
      | fprintf('','COMMENT: end icon text');
  "FIR Compiler 6.3 " : S-Function  LoadFcn=xlBlockLoadCallback(gcbh);  FunctionName=sysgen  Parameters=ptable_  EnableBusSupport=off  mask(Xilinx FIR Compiler 6.3 Block){coefficientvector=[6,0,-4,-3,5,6,-6,-13,7,44,64,44,7,-13,-6,6,5,-3,-4,0,6], coefficient_sets=1, coefficient_reload=off, filter_type=Single_Rate, rate_change_type=Integer, interpolation_rate=1, decimation_rate=1, zero_pack_factor=1, channel_sequence=Basic, number_channels=1, pattern_list='P4-0,P4-1,P4-2,P4-3,P4-4', number_paths=1, infoedit=Maximum Possible : Maximizes oversampling rate. Abstracted input handshake (no s_data_tvalid) and automatic rate propagation.<br>Hardware Oversampling Rate : Specifies oversampling rate relative to the input sample period. Abstracted input handshake (no s_data_tvalid) and automatic rate propagation.<br>Sample Period : Specifies absolute oversampling rate. No input handshake abstraction (exposes s_data_tvalid) and no rate propagation., ratespecification=Maximum_Possible, sampleperiod=1, hardwareoversamplingrate=1, coefficient_sign=Signed, quantization=Integer_Coefficients, coefficient_width=16, bestprecision=on, coefficient_fractional_bits=0, coefficient_structure=Inferred, output_rounding_mode=Full_Precision, output_width=24, xl_use_area=off, xl_area=[0,0,0,0,0,0,0], filter_architecture=Systolic_Multiply_Accumulate, optimization_goal=Area, data_buffer_type=Automatic, coefficient_buffer_type=Automatic, input_buffer_type=Automatic, output_buffer_type=Automatic, preference_for_other_storage=Automatic, multi_column_support=Automatic, columnconfig='1', inter_column_pipe_length=4, data_has_tlast=Not_Required, m_data_has_tready=off, s_data_has_fifo=off, s_data_has_tuser=Not_Required, m_data_has_tuser=Not_Required, s_config_sync_mode=On_Vector, s_config_method=Single, num_reload_slots=1, has_aclken=off, has_aresetn=off, infoeditControl=ARESETn must be asserted for a minmum of 2 cycles, trim_axipin_name=on, passband_min=0.0, passband_max=0.5, stopband_min=0.5, stopband_max=1.0, filter_selection=1, gui_behaviour=Sysgen_GUI, data_sign=Signed, data_width=16, data_fractional_bits=0, data_tuser_width=1, wrapper_available=true, ip_wrap_arbitrary_binary_point=true, simulation_type=external_xfix, simulation_model=firv6_3_CModel:firv6_3_cmodel, ip_name=FIR Compiler, ip_version=6.3, dsptool_ready=true, ipcore_usecache=true, ipcore_useipmodelcache=true, ipcore_xco_need_fpga_part=true, port_translation_map={ 'aclken' => 'en', 'aresetn' => 'rst' }, run_core_at_system_period=true, ipcore_fpga_part=xlipgetpartsetting(gcb, {'virtex6', 'xc6vlx75t', '-3', 'ff784'}), has_advanced_control=0, sggui_pos=-1,-1,-1,-1, block_type=fir_compiler_v6_3, block_version=, sg_icon_stat=240,206,1,3,white,blue,0,f63fefcf,right,,[2 ],[2 3 3 ], sg_mask_display=|, sg_list_contents=, sg_blockgui_xml=}
      mask sg_mask_display=|
      | fprintf('','COMMENT: begin icon graphics');
      | patch([0 0 4 4 ],[172 34 34 172 ],[5.466667e-001 5.800000e-001 6.400000e-001 ]);
      | patch([236 236 240 240 ],[197 149 149 197 ],[5.466667e-001 5.800000e-001 6.400000e-001 ]);
      | patch([236 236 240 240 ],[127 9 9 127 ],[3.233333e-001 3.400000e-001 3.700000e-001 ]);
      | patch([4 235 235 4 4 ],[0 0 206 206 0 ],[7.700000e-001 8.200000e-001 9.100000e-001 ]);
      | plot([4 235 235 4 4 ],[0 0 206 206 0 ]);
      |
      |
      | patch([55.475 97.38 126.38 155.38 184.38 126.38 84.475 55.475 ],[135.19 135.19 164.19 135.19 164.19 164.19 164.19 135.19 ],[1 1 1 ]);
      | patch([84.475 126.38 97.38 55.475 84.475 ],[106.19 106.19 135.19 135.19 106.19 ],[0.931 0.946 0.973 ]);
      | patch([55.475 97.38 126.38 84.475 55.475 ],[77.19 77.19 106.19 106.19 77.19 ],[1 1 1 ]);
      | patch([84.475 184.38 155.38 126.38 97.38 55.475 84.475 ],[48.19 48.19 77.19 48.19 77.19 77.19 48.19 ],[0.931 0.946 0.973 ]);
      | fprintf('','COMMENT: end icon graphics');
      | fprintf('','COMMENT: begin icon text');
      | color('black');port_label('input',1,'  data_tdata  ');
      | color('black');port_label('output',1,'  data_tready  ');
      | color('black');port_label('output',2,'  data_tvalid  ');
      | color('black');port_label('output',3,'  data_tdata  ');
      | fprintf('','COMMENT: end icon text');
      mask prompts: coefficientvector "Coefficient Vector :"; coefficient_sets "Number of Coefficient Sets :"; coefficient_reload "Use Reloadable Coefficients"; filter_type "Filter Type :"; rate_change_type "Rate Change Type :"; interpolation_rate "Interpolation Rate Value :"; decimation_rate "Decimation Rate Value :"; zero_pack_factor "Zero Pack Factor :"; channel_sequence "Channel Sequence :"; number_channels "Number of Channels :"; pattern_list "Sequence ID List :"; number_paths "Number of Paths :"; infoedit ""; ratespecification "Select format :"; sampleperiod "Sample period :"; hardwareoversamplingrate "Hardware Oversampling Rate :"; coefficient_sign "Coefficient Type :"; quantization "Quantization :"; coefficient_width "Coefficient Width :"; bestprecision "Best Precision Fraction Length"; coefficient_fractional_bits "Coefficient Fractional Bits :"; coefficient_structure "Coefficient Structure :"; output_rounding_mode "Output Rounding Mode :"; output_width "Output Width :"; xl_use_area "Define FPGA area for resource estimation"; xl_area "FPGA area [slices, FFs, BRAMs, LUTs, IOBs, emb. mults, TBUFs]"; filter_architecture "Filter Architecture :"; optimization_goal "Optimization Goal"; data_buffer_type "Data Buffer Type :"; coefficient_buffer_type "Coefficient Buffer Type :"; input_buffer_type "Input Buffer Type :"; output_buffer_type "Output Buffer Type :"; preference_for_other_storage "Preference for other storage :"; multi_column_support "Multi-Column Support :"; columnconfig "Column Configuration :"; inter_column_pipe_length "Inter-Column Pipe Length :"; data_has_tlast "TLAST"; m_data_has_tready "Output TREADY"; s_data_has_fifo "Input FIFO"; s_data_has_tuser "Input :"; m_data_has_tuser "Output :"; s_config_sync_mode "Synchronization Mode :"; s_config_method "Configuration Method :"; num_reload_slots "Reload Slots"; has_aclken "ACLKEN"; has_aresetn "ARESETn (active low)"; infoeditControl ""; trim_axipin_name "Display shortened port names"; passband_min ""; passband_max ""; stopband_min ""; stopband_max ""; filter_selection ""; gui_behaviour ""; data_sign ""; data_width ""; data_fractional_bits ""; data_tuser_width ""; wrapper_available ""; ip_wrap_arbitrary_binary_point ""; simulation_type ""; simulation_model ""; ip_name ""; ip_version ""; dsptool_ready ""; ipcore_usecache ""; ipcore_useipmodelcache ""; ipcore_xco_need_fpga_part ""; port_translation_map ""; run_core_at_system_period ""; ipcore_fpga_part ""; has_advanced_control ""; sggui_pos ""; block_type ""; block_version ""; sg_icon_stat ""; sg_mask_display ""; sg_list_contents ""; sg_blockgui_xml ""
      mask help:
      | Maximum Possible : Maximizes oversampling rate. Abstracted input handshake (no s_data_tvalid) and automatic rate propagation.
      | Hardware Oversampling Rate : Specifies oversampling rate relative to the input sample period. Abstracted input handshake (no s_data_tvalid) and automatic rate propagation.
      | Sample Period : Specifies absolute oversampling rate. No input handshake abstraction (exposes s_data_tvalid) and no rate propagation.
      mask init:
      | try
      |   tmp_gcb = gcb;
      |   tmp_gcbh = gcbh;
      |   if (strcmp('SysGenIndex',get_param(bdroot(tmp_gcbh),'tag')) && ~isempty(regexp(bdroot(tmp_gcb), '^xbs', 'once')))
      |     return;
      |   end;
      |   xlMungeMaskParams;
      |   block_config = 'sysgen:coregenimport_config';
      | 
      |   block_type='fir_compiler_v6_3';
      | 
      |   serialized_declarations = '{''bestprecision''=>''Bool'',''channel_sequence''=>''String'',''coefficient_buffer_type''=>''String'',''coefficient_fractional_bits''=>''Int'',''coefficient_reload''=>''Bool'',''coefficient_sets''=>''Int'',''coefficient_sign''=>''String'',''coefficient_structure''=>''String'',''coefficient_width''=>''Int'',''coefficientvector''=>''DoubleVector'',''columnconfig''=>''String'',''data_buffer_type''=>''String'',''data_fractional_bits''=>''Int'',''data_has_tlast''=>''String'',''data_sign''=>''String'',''data_tuser_width''=>''Int'',''data_width''=>''Int'',''decimation_rate''=>''Int'',''dsptool_ready''=>''Bool'',''filter_architecture''=>''String'',''filter_selection''=>''Int'',''filter_type''=>''String'',''gui_behaviour''=>''String'',''hardwareoversamplingrate''=>''Int'',''has_aclken''=>''Bool'',''has_aresetn''=>''Bool'',''input_buffer_type''=>''String'',''inter_column_pipe_length''=>''Int'',''interpolation_rate''=>''Int'',''ip_name''=>''String'',''ip_version''=>''String'',''ip_wrap_arbitrary_binary_point''=>''Bool'',''ipcore_fpga_part''=>''StringVector'',''ipcore_usecache''=>''Bool'',''ipcore_useipmodelcache''=>''Bool'',''ipcore_xco_need_fpga_part''=>''Bool'',''m_data_has_tready''=>''Bool'',''m_data_has_tuser''=>''String'',''multi_column_support''=>''String'',''num_reload_slots''=>''Int'',''number_channels''=>''Int'',''number_paths''=>''Int'',''optimization_goal''=>''String'',''output_buffer_type''=>''String'',''output_rounding_mode''=>''String'',''output_width''=>''Int'',''passband_max''=>''Double'',''passband_min''=>''Double'',''pattern_list''=>''String'',''port_translation_map''=>''String'',''preference_for_other_storage''=>''String'',''quantization''=>''String'',''rate_change_type''=>''String'',''ratespecification''=>''String'',''run_core_at_system_period''=>''Bool'',''s_config_method''=>''String'',''s_config_sync_mode''=>''String'',''s_data_has_fifo''=>''Bool'',''s_data_has_tuser''=>''String'',''sampleperiod''=>''Int'',''simulation_model''=>''String'',''simulation_type''=>''String'',''stopband_max''=>''Double'',''stopband_min''=>''Double'',''trim_axipin_name''=>''Int'',''wrapper_available''=>''Bool'',''xl_use_area''=>''Bool'',''zero_pack_factor''=>''Int'',''block_type''=>''String''}';
      |   ptable_ = xlblockprep(get_param(tmp_gcb, 'MaskWSVariables'));
      |   try
      |     xlBlockMoveCallback(tmp_gcbh);
      |   catch 
      |      clear global xl_updateicon_recursion_guard;
      |   end;
      | catch
      |   global dbgsysgen;
      |   if(~isempty(dbgsysgen) && dbgsysgen)
      |     e = regexprep(lasterr, '\n', '\nError: ');
      |     disp(['Error: While running MaskInit code on block ' tmp_gcb ': ' e]);
      |     error(e);
      |   end
      | end
      settings: CopyFcn=xlBlockMoveCallback(gcbh);  DeleteFcn=xlDestroyGui(gcbh);  ModelCloseFcn=xlDestroyGui(gcbh);  PreSaveFcn=xlBlockPreSaveCallback(gcbh);  PostSaveFcn=xlBlockPostSaveCallback(gcbh);  DestroyFcn=xlDestroyGui(gcbh);  OpenFcn=xlOpenGui(gcbh, 'fir_compiler_v6_3_gui.xml', @xlipmagiccallback_pass_evaluate_params, @fir_compiler_v6_3_action)  CloseFcn=xlDestroyGui(gcbh);  MoveFcn=xlBlockMoveCallback(gcbh);
      mask Help: eval('');xlDoc('-book','sysgen','-topic','FIR_Compiler_6_3');
      mask StyleString: edit,edit,checkbox,popup(Single_Rate|Interpolation|Decimation|Hilbert|Interpolated),popup(Integer|Fixed_Fractional),edit,edit,edit,popup(Basic|Advanced),edit,edit,edit,edit,popup(Maximum_Possible|Sample_Period|Hardware_Oversampling_Rate),edit,edit,popup(Signed|Unsigned),popup(Integer_Coefficients|Quantize_Only|Maximize_Dynamic_Range),edit,checkbox,edit,popup(Inferred|Non_Symmetric|Symmetric|Negative_Symmetric|Half_Band|Hilbert),popup(Full_Precision|Truncate_LSBs|Non_Symmetric_Rounding_Down|Non_Symmetric_Rounding_Up|Symmetric_Rounding_to_Zero|Symmetric_Rounding_to_Infinity|Convergent_Rounding_to_Even|Convergent_Rounding_to_Odd),edit,checkbox,edit,popup(Systolic_Multiply_Accumulate|Transpose_Multiply_Accumulate),popup(Area|Speed|Speed_(Control_only)|Speed_(Data_only)),popup(Automatic|Block|Distributed|Not_Applicable),popup(Automatic|Block|Distributed|Not_Applicable),popup(Automatic|Block|Distributed|Not_Applicable),popup(Automatic|Block|Distributed|Not_Applicable),popup(Automatic|Block|Distributed|Not_Applicable),popup(Automatic|Custom),edit,edit,popup(Not_Required|Vector_Framing|Packet_Framing),checkbox,checkbox,popup(Not_Required|User_Field|Chan_ID_Field|User_and_Chan_ID_Field),popup(Not_Required|User_Field|Chan_ID_Field|User_and_Chan_ID_Field),popup(On_Vector|On_Packet),popup(Single|By_Channel),edit,checkbox,checkbox,edit,checkbox,edit,edit,edit,edit,edit,edit,edit,edit,edit,edit,edit,edit,edit,edit,edit,edit,edit,edit,edit,edit,edit,edit,edit,edit,edit,edit,edit,edit,edit,edit,edit
      mask Display:
      | fprintf('','COMMENT: begin icon graphics');
      | patch([0 0 4 4 ],[172 34 34 172 ],[5.466667e-001 5.800000e-001 6.400000e-001 ]);
      | patch([236 236 240 240 ],[197 149 149 197 ],[5.466667e-001 5.800000e-001 6.400000e-001 ]);
      | patch([236 236 240 240 ],[127 9 9 127 ],[3.233333e-001 3.400000e-001 3.700000e-001 ]);
      | patch([4 235 235 4 4 ],[0 0 206 206 0 ],[7.700000e-001 8.200000e-001 9.100000e-001 ]);
      | plot([4 235 235 4 4 ],[0 0 206 206 0 ]);
      | 
      | 
      | patch([55.475 97.38 126.38 155.38 184.38 126.38 84.475 55.475 ],[135.19 135.19 164.19 135.19 164.19 164.19 164.19 135.19 ],[1 1 1 ]);
      | patch([84.475 126.38 97.38 55.475 84.475 ],[106.19 106.19 135.19 135.19 106.19 ],[0.931 0.946 0.973 ]);
      | patch([55.475 97.38 126.38 84.475 55.475 ],[77.19 77.19 106.19 106.19 77.19 ],[1 1 1 ]);
      | patch([84.475 184.38 155.38 126.38 97.38 55.475 84.475 ],[48.19 48.19 77.19 48.19 77.19 77.19 48.19 ],[0.931 0.946 0.973 ]);
      | fprintf('','COMMENT: end icon graphics');
      | fprintf('','COMMENT: begin icon text');
      | color('black');port_label('input',1,'  data_tdata  ');
      | color('black');port_label('output',1,'  data_tready  ');
      | color('black');port_label('output',2,'  data_tvalid  ');
      | color('black');port_label('output',3,'  data_tdata  ');
      | fprintf('','COMMENT: end icon text');
  "FIR Compiler v1_0 " : S-Function  LoadFcn=xlBlockLoadCallback(gcbh);  FunctionName=sysgen  Parameters=ptable_  EnableBusSupport=off  mask(Xilinx FIR Compiler v1_0 Block){infoedit=Implements a high-speed multi-channel FIR filter.<br><br>Hardware  notes: Implemented using DSP48s hence only Virtex 4 supported., u_fir_type_sgadvanced=, u_fir_type=SingleRate, u_rate_change=1, u_channels=1, u_clks_samp=1, u_coefs=[1 2 3], u_coef_arith_sgadvanced=, u_coef_arith=Signed, u_coef_bits=16, u_coef_point=8, u_coef_struct_sgadvanced=, u_coef_struct=Inferred from Coefficients, u_display_info_sgadvanced=, u_display_info=off, u_valid_ports_sgadvanced=, u_valid_ports=off, u_en_port_sgadvanced=, u_en_port=off, u_core_rdy_port_sgadvanced=, u_core_rdy_port=off, u_rst_rfd_port_sgadvanced=, u_rst_rfd_port=off, dbl_ovrd_sgadvanced=, dbl_ovrd=off, u_storage_sgadvanced=, u_storage=Automatic, u_data_buf_sgadvanced=, u_data_buf=dist_mem, u_coef_buf_sgadvanced=, u_coef_buf=dist_mem, u_v4_options_sgadvanced=, u_v4_options=Disabled, u_xcol_pipe_sgadvanced=, u_xcol_pipe=1, u_first_length=1, u_wrap_length=1, xl_use_area_sgadvanced=, xl_use_area=off, xl_area=[0,0,0,0,0,0,0], u_coef_rows=1, u_coef_cols=3, u_coef_sets=1, u_coef_type=1, u_latency=1, enable_debug=0, has_advanced_control=0, sggui_pos=-1,-1,-1,-1, block_type=simple_fir, block_version=, sg_icon_stat=90,134,-1,-1,white,blue,0,07734,right,,[ ],[ ], sg_mask_display=|, sg_list_contents=, sg_blockgui_xml=}
      mask sg_mask_display=|
      | fprintf('','COMMENT: begin icon graphics');
      | patch([0 90 90 0 0 ],[0 0 134 134 0 ],[0.77 0.82 0.91 ]);
      | plot([0 90 90 0 0 ],[0 0 134 134 0 ]);
      | patch([18.3 35.64 47.64 59.64 71.64 47.64 30.3 18.3 ],[80.32 80.32 92.32 80.32 92.32 92.32 92.32 80.32 ],[1 1 1 ]);
      | patch([30.3 47.64 35.64 18.3 30.3 ],[68.32 68.32 80.32 80.32 68.32 ],[0.931 0.946 0.973 ]);
      | patch([18.3 35.64 47.64 30.3 18.3 ],[56.32 56.32 68.32 68.32 56.32 ],[1 1 1 ]);
      | patch([30.3 71.64 59.64 47.64 35.64 18.3 30.3 ],[44.32 44.32 56.32 44.32 56.32 56.32 44.32 ],[0.931 0.946 0.973 ]);
      | fprintf('','COMMENT: end icon graphics');
      | fprintf('','COMMENT: begin icon text');
      | fprintf('','COMMENT: end icon text');
      mask prompts: infoedit ""; u_fir_type_sgadvanced ""; u_fir_type "Filter type"; u_rate_change "Sample rate change"; u_channels "Number of channels"; u_clks_samp "Hardware over-sampling rate"; u_coefs "Coefficient vector"; u_coef_arith_sgadvanced ""; u_coef_arith "Arithmetic type"; u_coef_bits "Number of bits"; u_coef_point "Binary point"; u_coef_struct_sgadvanced ""; u_coef_struct "Structure"; u_display_info_sgadvanced ""; u_display_info "Display filter information on block icon"; u_valid_ports_sgadvanced ""; u_valid_ports "Provide valid ports"; u_en_port_sgadvanced ""; u_en_port "Provide <tt>en</tt> port"; u_core_rdy_port_sgadvanced ""; u_core_rdy_port "Provide <tt>core_rdy</tt> port"; u_rst_rfd_port_sgadvanced ""; u_rst_rfd_port "Provide <tt>rst</tt> and <tt>rfd</tt> ports"; dbl_ovrd_sgadvanced ""; dbl_ovrd "Override with doubles"; u_storage_sgadvanced ""; u_storage ""; u_data_buf_sgadvanced ""; u_data_buf "Data buffer"; u_coef_buf_sgadvanced ""; u_coef_buf "Coefficient buffer"; u_v4_options_sgadvanced ""; u_v4_options ""; u_xcol_pipe_sgadvanced ""; u_xcol_pipe "Cross column pipelining"; u_first_length "First column length"; u_wrap_length "Column wrap length"; xl_use_area_sgadvanced ""; xl_use_area "Define FPGA area for resource estimation"; xl_area "FPGA area [slices, FFs, BRAMs, LUTs, IOBs, emb. mults, TBUFs]"; u_coef_rows ""; u_coef_cols ""; u_coef_sets ""; u_coef_type ""; u_latency ""; enable_debug ""; has_advanced_control ""; sggui_pos ""; block_type ""; block_version ""; sg_icon_stat ""; sg_mask_display ""; sg_list_contents ""; sg_blockgui_xml ""
      mask help:
      | Implements a high-speed multi-channel FIR filter.
      |
      | Hardware  notes: Implemented using DSP48s hence only Virtex 4 supported.
      mask init:
      | try
      |   tmp_gcb = gcb;
      |   tmp_gcbh = gcbh;
      |   if (strcmp('SysGenIndex',get_param(bdroot(tmp_gcbh),'tag')) && ~isempty(regexp(bdroot(tmp_gcb), '^xbs', 'once')))
      |     return;
      |   end;
      |   xlMungeMaskParams;
      |   block_config = 'sysgen_blockset:Removed_config';
      | 
      |   block_type='simple_fir';
      | nport = get_param(gcbh, 'ports');
      | nin = nport(1);
      | nout = nport(2);
      | 
      |   serialized_declarations = '{''enable_debug''=>''Int'',''u_channels''=>''Int'',''u_clks_samp''=>''Int'',''u_coef_arith''=>''Int'',''u_coef_bits''=>''Int'',''u_coef_buf''=>''Int'',''u_coef_cols''=>''Int'',''u_coef_point''=>''Int'',''u_coef_rows''=>''Int'',''u_coef_sets''=>''Int'',''u_coef_struct''=>''Int'',''u_coef_type''=>''Int'',''u_coefs''=>''DoubleVector'',''u_core_rdy_port''=>''Int'',''u_data_buf''=>''Int'',''u_display_info''=>''Int'',''u_en_port''=>''Int'',''u_fir_type''=>''Int'',''u_first_length''=>''Int'',''u_latency''=>''Int'',''u_rate_change''=>''Int'',''u_rst_rfd_port''=>''Int'',''u_storage''=>''Int'',''u_v4_options''=>''Int'',''u_valid_ports''=>''Int'',''u_wrap_length''=>''Int'',''u_xcol_pipe''=>''Int'',''block_type''=>''String'',''nin''=>''Double'',''nout''=>''Double''}';
      |   xlsimple_fir_init();
      |   ptable_ = xlblockprep(get_param(tmp_gcb, 'MaskWSVariables'));
      |   try
      |     xlBlockMoveCallback(tmp_gcbh);
      |   catch 
      |      clear global xl_updateicon_recursion_guard;
      |   end;
      | catch
      |   global dbgsysgen;
      |   if(~isempty(dbgsysgen) && dbgsysgen)
      |     e = regexprep(lasterr, '\n', '\nError: ');
      |     disp(['Error: While running MaskInit code on block ' tmp_gcb ': ' e]);
      |     error(e);
      |   end
      | end
      settings: CopyFcn=xlBlockMoveCallback(gcbh);  DeleteFcn=xlDestroyGui(gcbh);  ModelCloseFcn=xlDestroyGui(gcbh);  PreSaveFcn=xlBlockPreSaveCallback(gcbh);  PostSaveFcn=xlBlockPostSaveCallback(gcbh);  DestroyFcn=xlDestroyGui(gcbh);  OpenFcn=xlOpenGui(gcbh, 'simple_fir_gui.xml', @xlremovedenablement, -1)  CloseFcn=xlDestroyGui(gcbh);  MoveFcn=xlBlockMoveCallback(gcbh);
      mask Help: eval('');xlDoc('-book','sysgen','-topic','FIR_Compiler_v1_0');
      mask StyleString: edit,edit,popup(SingleRate|Decimation|Interpolation),edit,edit,edit,edit,edit,popup(Signed|Unsigned),edit,edit,edit,popup(Inferred from Coefficients|Non-Symmetric|Symmetric|Negative-Symmetric|Half Band),edit,checkbox,edit,checkbox,edit,checkbox,edit,checkbox,edit,checkbox,edit,checkbox,edit,popup(Automatic|Custom),edit,popup(dist_mem|block_mem),edit,popup(dist_mem|block_mem),edit,popup(Disabled|Custom),edit,popup(1|2|3|4|5|6|7|8|9|10|11|12|13|14|15|16),edit,edit,edit,checkbox,edit,edit,edit,edit,edit,edit,edit,edit,edit,edit,edit,edit,edit,edit,edit
      mask Display:
      | fprintf('','COMMENT: begin icon graphics');
      | patch([0 90 90 0 0 ],[0 0 134 134 0 ],[0.77 0.82 0.91 ]);
      | plot([0 90 90 0 0 ],[0 0 134 134 0 ]);
      | patch([18.3 35.64 47.64 59.64 71.64 47.64 30.3 18.3 ],[80.32 80.32 92.32 80.32 92.32 92.32 92.32 80.32 ],[1 1 1 ]);
      | patch([30.3 47.64 35.64 18.3 30.3 ],[68.32 68.32 80.32 80.32 68.32 ],[0.931 0.946 0.973 ]);
      | patch([18.3 35.64 47.64 30.3 18.3 ],[56.32 56.32 68.32 68.32 56.32 ],[1 1 1 ]);
      | patch([30.3 71.64 59.64 47.64 35.64 18.3 30.3 ],[44.32 44.32 56.32 44.32 56.32 56.32 44.32 ],[0.931 0.946 0.973 ]);
      | fprintf('','COMMENT: end icon graphics');
      | fprintf('','COMMENT: begin icon text');
      | fprintf('','COMMENT: end icon text');
  "FIR Compiler v2_0 " : S-Function  LoadFcn=xlBlockLoadCallback(gcbh);  FunctionName=sysgen  Parameters=ptable_  EnableBusSupport=off  mask(Xilinx FIR Compiler v2_0 Block){infoedit=Implements a high-speed multi-channel FIR filter.<br><br>Hardware  notes: Implemented using DSP48s hence only Virtex 4 and Virtex 5 devices are supported., u_fir_type_sgadvanced=, u_fir_type=SingleRate, u_rate_change=1, u_channels=1, u_clks_samp=1, u_coefs=[1 2 3], u_coef_arith_sgadvanced=, u_coef_arith=Signed, u_coef_bits=16, u_coef_point=8, u_coef_struct_sgadvanced=, u_coef_struct=Inferred from Coefficients, reload_coef_sgadvanced=, reload_coef=off, u_display_info_sgadvanced=, u_display_info=off, u_valid_ports_sgadvanced=, u_valid_ports=off, u_en_port_sgadvanced=, u_en_port=off, u_core_rdy_port_sgadvanced=, u_core_rdy_port=off, u_rst_rfd_port_sgadvanced=, u_rst_rfd_port=off, dbl_ovrd_sgadvanced=, dbl_ovrd=off, u_storage_sgadvanced=, u_storage=Automatic, u_data_buf_sgadvanced=, u_data_buf=dist_mem, u_coef_buf_sgadvanced=, u_coef_buf=dist_mem, u_v4_options_sgadvanced=, u_v4_options=Disabled, u_xcol_pipe_sgadvanced=, u_xcol_pipe=4, u_first_length=32, u_wrap_length=32, xl_use_area_sgadvanced=, xl_use_area=off, xl_area=[0,0,0,0,0,0,0], u_coef_rows=1, u_coef_cols=3, u_coef_sets=1, u_coef_type=1, u_latency=1, enable_debug=0, has_advanced_control=0, sggui_pos=-1,-1,-1,-1, block_type=Fir_compiler_v2_0, block_version=, sg_icon_stat=90,134,-1,-1,white,blue,0,07734,right,,[ ],[ ], sg_mask_display=|, sg_list_contents=, sg_blockgui_xml=}
      mask sg_mask_display=|
      | fprintf('','COMMENT: begin icon graphics');
      | patch([0 90 90 0 0 ],[0 0 134 134 0 ],[0.77 0.82 0.91 ]);
      | plot([0 90 90 0 0 ],[0 0 134 134 0 ]);
      | patch([18.3 35.64 47.64 59.64 71.64 47.64 30.3 18.3 ],[80.32 80.32 92.32 80.32 92.32 92.32 92.32 80.32 ],[1 1 1 ]);
      | patch([30.3 47.64 35.64 18.3 30.3 ],[68.32 68.32 80.32 80.32 68.32 ],[0.931 0.946 0.973 ]);
      | patch([18.3 35.64 47.64 30.3 18.3 ],[56.32 56.32 68.32 68.32 56.32 ],[1 1 1 ]);
      | patch([30.3 71.64 59.64 47.64 35.64 18.3 30.3 ],[44.32 44.32 56.32 44.32 56.32 56.32 44.32 ],[0.931 0.946 0.973 ]);
      | fprintf('','COMMENT: end icon graphics');
      | fprintf('','COMMENT: begin icon text');
      | fprintf('','COMMENT: end icon text');
      mask prompts: infoedit ""; u_fir_type_sgadvanced ""; u_fir_type "Filter type"; u_rate_change "Sample rate change"; u_channels "Number of channels"; u_clks_samp "Hardware over-sampling rate"; u_coefs "Coefficient vector"; u_coef_arith_sgadvanced ""; u_coef_arith "Arithmetic type"; u_coef_bits "Number of bits"; u_coef_point "Binary point"; u_coef_struct_sgadvanced ""; u_coef_struct "Structure"; reload_coef_sgadvanced ""; reload_coef "Use reloadable coefficients"; u_display_info_sgadvanced ""; u_display_info "Display filter information on block icon"; u_valid_ports_sgadvanced ""; u_valid_ports "Provide valid ports"; u_en_port_sgadvanced ""; u_en_port "Provide <tt>en</tt> port"; u_core_rdy_port_sgadvanced ""; u_core_rdy_port "Provide <tt>core_rdy</tt> port"; u_rst_rfd_port_sgadvanced ""; u_rst_rfd_port "Provide <tt>rst</tt> and <tt>rfd</tt> ports"; dbl_ovrd_sgadvanced ""; dbl_ovrd "Override with doubles"; u_storage_sgadvanced ""; u_storage ""; u_data_buf_sgadvanced ""; u_data_buf "Data buffer"; u_coef_buf_sgadvanced ""; u_coef_buf "Coefficient buffer"; u_v4_options_sgadvanced ""; u_v4_options ""; u_xcol_pipe_sgadvanced ""; u_xcol_pipe "Cross column pipelining"; u_first_length "First column length"; u_wrap_length "Column wrap length"; xl_use_area_sgadvanced ""; xl_use_area "Define FPGA area for resource estimation"; xl_area "FPGA area [slices, FFs, BRAMs, LUTs, IOBs, emb. mults, TBUFs]"; u_coef_rows ""; u_coef_cols ""; u_coef_sets ""; u_coef_type ""; u_latency ""; enable_debug ""; has_advanced_control ""; sggui_pos ""; block_type ""; block_version ""; sg_icon_stat ""; sg_mask_display ""; sg_list_contents ""; sg_blockgui_xml ""
      mask help:
      | Implements a high-speed multi-channel FIR filter.
      |
      | Hardware  notes: Implemented using DSP48s hence only Virtex 4 and Virtex 5 devices are supported.
      mask init:
      | try
      |   tmp_gcb = gcb;
      |   tmp_gcbh = gcbh;
      |   if (strcmp('SysGenIndex',get_param(bdroot(tmp_gcbh),'tag')) && ~isempty(regexp(bdroot(tmp_gcb), '^xbs', 'once')))
      |     return;
      |   end;
      |   xlMungeMaskParams;
      |   block_config = 'sysgen_blockset:Removed_config';
      | 
      |   block_type='Fir_compiler_v2_0';
      | nport = get_param(gcbh, 'ports');
      | nin = nport(1);
      | nout = nport(2);
      | 
      |   serialized_declarations = '{''enable_debug''=>''Int'',''reload_coef''=>''Int'',''u_channels''=>''Int'',''u_clks_samp''=>''Int'',''u_coef_arith''=>''Int'',''u_coef_bits''=>''Int'',''u_coef_buf''=>''Int'',''u_coef_cols''=>''Int'',''u_coef_point''=>''Int'',''u_coef_rows''=>''Int'',''u_coef_sets''=>''Int'',''u_coef_struct''=>''Int'',''u_coef_type''=>''Int'',''u_coefs''=>''DoubleVector'',''u_core_rdy_port''=>''Int'',''u_data_buf''=>''Int'',''u_display_info''=>''Int'',''u_en_port''=>''Int'',''u_fir_type''=>''Int'',''u_first_length''=>''Int'',''u_latency''=>''Int'',''u_rate_change''=>''Int'',''u_rst_rfd_port''=>''Int'',''u_storage''=>''Int'',''u_v4_options''=>''Int'',''u_valid_ports''=>''Int'',''u_wrap_length''=>''Int'',''u_xcol_pipe''=>''Int'',''block_type''=>''String'',''nin''=>''Double'',''nout''=>''Double''}';
      |   xlFir_compiler_v2_0_init();
      |   ptable_ = xlblockprep(get_param(tmp_gcb, 'MaskWSVariables'));
      |   try
      |     xlBlockMoveCallback(tmp_gcbh);
      |   catch 
      |      clear global xl_updateicon_recursion_guard;
      |   end;
      | catch
      |   global dbgsysgen;
      |   if(~isempty(dbgsysgen) && dbgsysgen)
      |     e = regexprep(lasterr, '\n', '\nError: ');
      |     disp(['Error: While running MaskInit code on block ' tmp_gcb ': ' e]);
      |     error(e);
      |   end
      | end
      settings: CopyFcn=xlBlockMoveCallback(gcbh);  DeleteFcn=xlDestroyGui(gcbh);  ModelCloseFcn=xlDestroyGui(gcbh);  PreSaveFcn=xlBlockPreSaveCallback(gcbh);  PostSaveFcn=xlBlockPostSaveCallback(gcbh);  DestroyFcn=xlDestroyGui(gcbh);  OpenFcn=xlOpenGui(gcbh, 'Fir_compiler_v2_0_gui.xml', @xlremovedenablement, -1)  CloseFcn=xlDestroyGui(gcbh);  MoveFcn=xlBlockMoveCallback(gcbh);
      mask Help: eval('');xlDoc('-book','sysgen','-topic','FIR_Compiler_v2_0');
      mask StyleString: edit,edit,popup(SingleRate|Decimation|Interpolation),edit,edit,edit,edit,edit,popup(Signed|Unsigned),edit,edit,edit,popup(Inferred from Coefficients|Non-Symmetric|Symmetric|Negative-Symmetric|Half Band),edit,checkbox,edit,checkbox,edit,checkbox,edit,checkbox,edit,checkbox,edit,checkbox,edit,checkbox,edit,popup(Automatic|Custom),edit,popup(dist_mem|block_mem),edit,popup(dist_mem|block_mem),edit,popup(Disabled|Custom),edit,popup(1|2|3|4|5|6|7|8|9|10|11|12|13|14|15|16),edit,edit,edit,checkbox,edit,edit,edit,edit,edit,edit,edit,edit,edit,edit,edit,edit,edit,edit,edit
      mask Display:
      | fprintf('','COMMENT: begin icon graphics');
      | patch([0 90 90 0 0 ],[0 0 134 134 0 ],[0.77 0.82 0.91 ]);
      | plot([0 90 90 0 0 ],[0 0 134 134 0 ]);
      | patch([18.3 35.64 47.64 59.64 71.64 47.64 30.3 18.3 ],[80.32 80.32 92.32 80.32 92.32 92.32 92.32 80.32 ],[1 1 1 ]);
      | patch([30.3 47.64 35.64 18.3 30.3 ],[68.32 68.32 80.32 80.32 68.32 ],[0.931 0.946 0.973 ]);
      | patch([18.3 35.64 47.64 30.3 18.3 ],[56.32 56.32 68.32 68.32 56.32 ],[1 1 1 ]);
      | patch([30.3 71.64 59.64 47.64 35.64 18.3 30.3 ],[44.32 44.32 56.32 44.32 56.32 56.32 44.32 ],[0.931 0.946 0.973 ]);
      | fprintf('','COMMENT: end icon graphics');
      | fprintf('','COMMENT: begin icon text');
      | fprintf('','COMMENT: end icon text');
  "FIR Compiler v3_0 " : S-Function  LoadFcn=xlBlockLoadCallback(gcbh);  FunctionName=sysgen  Parameters=ptable_  EnableBusSupport=off  mask(Xilinx FIR Compiler v3_0 Block){infoedit=Implements a high-speed multi-channel FIR filter.<br><br>Hardware  notes: Implemented using DSP48s hence only Virtex 4, Virtex 5 and SpartanDSP devices are supported., Filter_Type_sgadvanced=, Filter_Type=Single_Rate, Rate_Change=1, Zero_Pack_Factor=1, Number_Channels=1, Hardware_Oversampling=1, Coefficients=[1 2 3], Coefficient_Sign_sgadvanced=, Coefficient_Sign=Signed, Coefficient_Width=16, Coefficient_Binary_Point=8, Coefficient_Structure_sgadvanced=, Coefficient_Structure=Inferred, Coefficient_Reload_sgadvanced=, Coefficient_Reload=off, Display_Block_Info_sgadvanced=, Display_Block_Info=off, Valid_Ports_sgadvanced=, Valid_Ports=off, Enable_Port_sgadvanced=, Enable_Port=off, Rst_Rfd_Port_sgadvanced=, Rst_Rfd_Port=off, dbl_ovrd_sgadvanced=, dbl_ovrd=off, Storage_sgadvanced=, Storage=Automatic, Data_Buffer_Type_sgadvanced=, Data_Buffer_Type=Distributed, Coefficient_Buffer_Type_sgadvanced=, Coefficient_Buffer_Type=Distributed, Multiple_Column_Support_sgadvanced=, Multiple_Column_Support=Disabled, Inter_Column_Pipe_Length_sgadvanced=, Inter_Column_Pipe_Length=4, First_Column_Length=32, Column_Wrap_Length=32, xl_use_area_sgadvanced=, xl_use_area=off, xl_area=[0,0,0,0,0,0,0], u_coef_rows=1, u_coef_cols=3, u_coef_sets=1, u_coef_type=1, u_latency=1, enable_debug=0, has_advanced_control=0, sggui_pos=-1,-1,-1,-1, block_type=Fir_compiler_v3_0, block_version=, sg_icon_stat=90,134,-1,-1,white,blue,0,07734,right,,[ ],[ ], sg_mask_display=|, sg_list_contents=, sg_blockgui_xml=}
      mask sg_mask_display=|
      | fprintf('','COMMENT: begin icon graphics');
      | patch([0 90 90 0 0 ],[0 0 134 134 0 ],[0.77 0.82 0.91 ]);
      | plot([0 90 90 0 0 ],[0 0 134 134 0 ]);
      | patch([18.3 35.64 47.64 59.64 71.64 47.64 30.3 18.3 ],[80.32 80.32 92.32 80.32 92.32 92.32 92.32 80.32 ],[1 1 1 ]);
      | patch([30.3 47.64 35.64 18.3 30.3 ],[68.32 68.32 80.32 80.32 68.32 ],[0.931 0.946 0.973 ]);
      | patch([18.3 35.64 47.64 30.3 18.3 ],[56.32 56.32 68.32 68.32 56.32 ],[1 1 1 ]);
      | patch([30.3 71.64 59.64 47.64 35.64 18.3 30.3 ],[44.32 44.32 56.32 44.32 56.32 56.32 44.32 ],[0.931 0.946 0.973 ]);
      | fprintf('','COMMENT: end icon graphics');
      | fprintf('','COMMENT: begin icon text');
      | fprintf('','COMMENT: end icon text');
      mask prompts: infoedit ""; Filter_Type_sgadvanced ""; Filter_Type "Filter type"; Rate_Change "Sample rate change"; Zero_Pack_Factor "Zero Packing Factor"; Number_Channels "Number of channels"; Hardware_Oversampling "Hardware over-sampling rate"; Coefficients "Coefficient vector"; Coefficient_Sign_sgadvanced ""; Coefficient_Sign "Arithmetic type"; Coefficient_Width "Number of bits"; Coefficient_Binary_Point "Binary point"; Coefficient_Structure_sgadvanced ""; Coefficient_Structure "Structure"; Coefficient_Reload_sgadvanced ""; Coefficient_Reload "Use reloadable coefficients"; Display_Block_Info_sgadvanced ""; Display_Block_Info "Display filter information on block icon"; Valid_Ports_sgadvanced ""; Valid_Ports "Provide valid ports"; Enable_Port_sgadvanced ""; Enable_Port "Provide <tt>en</tt> port"; Rst_Rfd_Port_sgadvanced ""; Rst_Rfd_Port "Provide <tt>rst</tt> port"; dbl_ovrd_sgadvanced ""; dbl_ovrd "Override with doubles"; Storage_sgadvanced ""; Storage ""; Data_Buffer_Type_sgadvanced ""; Data_Buffer_Type "Data buffer"; Coefficient_Buffer_Type_sgadvanced ""; Coefficient_Buffer_Type "Coefficient buffer"; Multiple_Column_Support_sgadvanced ""; Multiple_Column_Support ""; Inter_Column_Pipe_Length_sgadvanced ""; Inter_Column_Pipe_Length "Cross column pipelining"; First_Column_Length "First column length"; Column_Wrap_Length "Column wrap length"; xl_use_area_sgadvanced ""; xl_use_area "Define FPGA area for resource estimation"; xl_area "FPGA area [slices, FFs, BRAMs, LUTs, IOBs, emb. mults, TBUFs]"; u_coef_rows ""; u_coef_cols ""; u_coef_sets ""; u_coef_type ""; u_latency ""; enable_debug ""; has_advanced_control ""; sggui_pos ""; block_type ""; block_version ""; sg_icon_stat ""; sg_mask_display ""; sg_list_contents ""; sg_blockgui_xml ""
      mask help:
      | Implements a high-speed multi-channel FIR filter.
      |
      | Hardware  notes: Implemented using DSP48s hence only Virtex 4, Virtex 5 and SpartanDSP devices are supported.
      mask init:
      | try
      |   tmp_gcb = gcb;
      |   tmp_gcbh = gcbh;
      |   if (strcmp('SysGenIndex',get_param(bdroot(tmp_gcbh),'tag')) && ~isempty(regexp(bdroot(tmp_gcb), '^xbs', 'once')))
      |     return;
      |   end;
      |   xlMungeMaskParams;
      |   block_config = 'sysgen_blockset:Removed_config';
      | 
      |   block_type='Fir_compiler_v3_0';
